simulink model "model"  (R2016a)
(part 3 of 3)

  bus36 : powerlib/Measurements/Load Flow Bus  LConnTagsString=a  Phases=single  Connectors=on one side  ID=bus36  Vbase=220000  Vref=1  Vangle=0  VLF=1  VLFb=1  VLFc=1  angleLF=0  angleLFb=0  angleLFc=0
      settings: AttributesFormatString=|
      | %<ID>
      | %<Vbase>V
      | %<VLF>pu
      | %<angleLF>deg.
      | %<Name>
  bus37 : powerlib/Measurements/Load Flow Bus  LConnTagsString=a  Phases=single  Connectors=on one side  ID=bus37  Vbase=220000  Vref=1  Vangle=0  VLF=1  VLFb=1  VLFc=1  angleLF=0  angleLFb=0  angleLFc=0
      settings: AttributesFormatString=|
      | %<ID>
      | %<Vbase>V
      | %<VLF>pu
      | %<angleLF>deg.
      | %<Name>
  bus38 : powerlib/Measurements/Load Flow Bus  LConnTagsString=a  Phases=single  Connectors=on one side  ID=bus38  Vbase=220000  Vref=1  Vangle=0  VLF=1  VLFb=1  VLFc=1  angleLF=0  angleLFb=0  angleLFc=0
      settings: AttributesFormatString=|
      | %<ID>
      | %<Vbase>V
      | %<VLF>pu
      | %<angleLF>deg.
      | %<Name>
  bus39 : powerlib/Measurements/Load Flow Bus  LConnTagsString=a  Phases=single  Connectors=on one side  ID=bus39  Vbase=220000  Vref=1  Vangle=0  VLF=1  VLFb=1  VLFc=1  angleLF=0  angleLFb=0  angleLFc=0
      settings: AttributesFormatString=|
      | %<ID>
      | %<Vbase>V
      | %<VLF>pu
      | %<angleLF>deg.
      | %<Name>
  bus4 : powerlib/Measurements/Load Flow Bus  LConnTagsString=a  Phases=single  Connectors=on one side  ID=bus4  Vbase=132000  Vref=1  Vangle=0  VLF=1  VLFb=1  VLFc=1  angleLF=0  angleLFb=0  angleLFc=0
      settings: AttributesFormatString=|
      | %<ID>
      | %<Vbase>V
      | %<VLF>pu
      | %<angleLF>deg.
      | %<Name>
  bus40 : powerlib/Measurements/Load Flow Bus  LConnTagsString=a  Phases=single  Connectors=on one side  ID=bus40  Vbase=220000  Vref=1  Vangle=0  VLF=1  VLFb=1  VLFc=1  angleLF=0  angleLFb=0  angleLFc=0
      settings: AttributesFormatString=|
      | %<ID>
      | %<Vbase>V
      | %<VLF>pu
      | %<angleLF>deg.
      | %<Name>
  bus41 : powerlib/Measurements/Load Flow Bus  LConnTagsString=a  Phases=single  Connectors=on one side  ID=bus41  Vbase=220000  Vref=1  Vangle=0  VLF=1  VLFb=1  VLFc=1  angleLF=0  angleLFb=0  angleLFc=0
      settings: AttributesFormatString=|
      | %<ID>
      | %<Vbase>V
      | %<VLF>pu
      | %<angleLF>deg.
      | %<Name>
  bus42 : powerlib/Measurements/Load Flow Bus  LConnTagsString=a  Phases=single  Connectors=on one side  ID=bus42  Vbase=220000  Vref=1  Vangle=0  VLF=1  VLFb=1  VLFc=1  angleLF=0  angleLFb=0  angleLFc=0
      settings: AttributesFormatString=|
      | %<ID>
      | %<Vbase>V
      | %<VLF>pu
      | %<angleLF>deg.
      | %<Name>
  bus43 : powerlib/Measurements/Load Flow Bus  LConnTagsString=a  Phases=single  Connectors=on one side  ID=bus43  Vbase=220000  Vref=1  Vangle=0  VLF=1  VLFb=1  VLFc=1  angleLF=0  angleLFb=0  angleLFc=0
      settings: AttributesFormatString=|
      | %<ID>
      | %<Vbase>V
      | %<VLF>pu
      | %<angleLF>deg.
      | %<Name>
  bus44 : powerlib/Measurements/Load Flow Bus  LConnTagsString=a  Phases=single  Connectors=on one side  ID=bus44  Vbase=220000  Vref=1  Vangle=0  VLF=1  VLFb=1  VLFc=1  angleLF=0  angleLFb=0  angleLFc=0
      settings: AttributesFormatString=|
      | %<ID>
      | %<Vbase>V
      | %<VLF>pu
      | %<angleLF>deg.
      | %<Name>
  bus45 : powerlib/Measurements/Load Flow Bus  LConnTagsString=a  Phases=single  Connectors=on one side  ID=bus45  Vbase=220000  Vref=1  Vangle=0  VLF=1  VLFb=1  VLFc=1  angleLF=0  angleLFb=0  angleLFc=0
      settings: AttributesFormatString=|
      | %<ID>
      | %<Vbase>V
      | %<VLF>pu
      | %<angleLF>deg.
      | %<Name>
  bus46 : powerlib/Measurements/Load Flow Bus  LConnTagsString=a  Phases=single  Connectors=on one side  ID=bus46  Vbase=220000  Vref=1  Vangle=0  VLF=1  VLFb=1  VLFc=1  angleLF=0  angleLFb=0  angleLFc=0
      settings: AttributesFormatString=|
      | %<ID>
      | %<Vbase>V
      | %<VLF>pu
      | %<angleLF>deg.
      | %<Name>
  bus47 : powerlib/Measurements/Load Flow Bus  LConnTagsString=a  Phases=single  Connectors=on one side  ID=bus47  Vbase=220000  Vref=1  Vangle=0  VLF=1  VLFb=1  VLFc=1  angleLF=0  angleLFb=0  angleLFc=0
      settings: AttributesFormatString=|
      | %<ID>
      | %<Vbase>V
      | %<VLF>pu
      | %<angleLF>deg.
      | %<Name>
  bus48 : powerlib/Measurements/Load Flow Bus  LConnTagsString=a  Phases=single  Connectors=on one side  ID=bus48  Vbase=220000  Vref=1  Vangle=0  VLF=1  VLFb=1  VLFc=1  angleLF=0  angleLFb=0  angleLFc=0
      settings: AttributesFormatString=|
      | %<ID>
      | %<Vbase>V
      | %<VLF>pu
      | %<angleLF>deg.
      | %<Name>
  bus49 : powerlib/Measurements/Load Flow Bus  LConnTagsString=a  Phases=single  Connectors=on one side  ID=bus49  Vbase=220000  Vref=1  Vangle=0  VLF=1  VLFb=1  VLFc=1  angleLF=0  angleLFb=0  angleLFc=0
      settings: AttributesFormatString=|
      | %<ID>
      | %<Vbase>V
      | %<VLF>pu
      | %<angleLF>deg.
      | %<Name>
  bus5 : powerlib/Measurements/Load Flow Bus  LConnTagsString=a  Phases=single  Connectors=on one side  ID=bus5  Vbase=132000  Vref=1  Vangle=0  VLF=1  VLFb=1  VLFc=1  angleLF=0  angleLFb=0  angleLFc=0
      settings: AttributesFormatString=|
      | %<ID>
      | %<Vbase>V
      | %<VLF>pu
      | %<angleLF>deg.
      | %<Name>
  bus50 : powerlib/Measurements/Load Flow Bus  LConnTagsString=a  Phases=single  Connectors=on one side  ID=bus50  Vbase=220000  Vref=1  Vangle=0  VLF=1  VLFb=1  VLFc=1  angleLF=0  angleLFb=0  angleLFc=0
      settings: AttributesFormatString=|
      | %<ID>
      | %<Vbase>V
      | %<VLF>pu
      | %<angleLF>deg.
      | %<Name>
  bus51 : powerlib/Measurements/Load Flow Bus  LConnTagsString=a  Phases=single  Connectors=on one side  ID=bus51  Vbase=220000  Vref=1  Vangle=0  VLF=1  VLFb=1  VLFc=1  angleLF=0  angleLFb=0  angleLFc=0
      settings: AttributesFormatString=|
      | %<ID>
      | %<Vbase>V
      | %<VLF>pu
      | %<angleLF>deg.
      | %<Name>
  bus52 : powerlib/Measurements/Load Flow Bus  LConnTagsString=a  Phases=single  Connectors=on one side  ID=bus52  Vbase=220000  Vref=1  Vangle=0  VLF=1  VLFb=1  VLFc=1  angleLF=0  angleLFb=0  angleLFc=0
      settings: AttributesFormatString=|
      | %<ID>
      | %<Vbase>V
      | %<VLF>pu
      | %<angleLF>deg.
      | %<Name>
  bus53 : powerlib/Measurements/Load Flow Bus  LConnTagsString=a  Phases=single  Connectors=on one side  ID=bus53  Vbase=220000  Vref=1  Vangle=0  VLF=1  VLFb=1  VLFc=1  angleLF=0  angleLFb=0  angleLFc=0
      settings: AttributesFormatString=|
      | %<ID>
      | %<Vbase>V
      | %<VLF>pu
      | %<angleLF>deg.
      | %<Name>
  bus54 : powerlib/Measurements/Load Flow Bus  LConnTagsString=a  Phases=single  Connectors=on one side  ID=bus54  Vbase=220000  Vref=1  Vangle=0  VLF=1  VLFb=1  VLFc=1  angleLF=0  angleLFb=0  angleLFc=0
      settings: AttributesFormatString=|
      | %<ID>
      | %<Vbase>V
      | %<VLF>pu
      | %<angleLF>deg.
      | %<Name>
  bus55 : powerlib/Measurements/Load Flow Bus  LConnTagsString=a  Phases=single  Connectors=on one side  ID=bus55  Vbase=220000  Vref=1  Vangle=0  VLF=1  VLFb=1  VLFc=1  angleLF=0  angleLFb=0  angleLFc=0
      settings: AttributesFormatString=|
      | %<ID>
      | %<Vbase>V
      | %<VLF>pu
      | %<angleLF>deg.
      | %<Name>
  bus56 : powerlib/Measurements/Load Flow Bus  LConnTagsString=a  Phases=single  Connectors=on one side  ID=bus56  Vbase=220000  Vref=1  Vangle=0  VLF=1  VLFb=1  VLFc=1  angleLF=0  angleLFb=0  angleLFc=0
      settings: AttributesFormatString=|
      | %<ID>
      | %<Vbase>V
      | %<VLF>pu
      | %<angleLF>deg.
      | %<Name>
  bus57 : powerlib/Measurements/Load Flow Bus  LConnTagsString=a  Phases=single  Connectors=on one side  ID=bus57  Vbase=220000  Vref=1  Vangle=0  VLF=1  VLFb=1  VLFc=1  angleLF=0  angleLFb=0  angleLFc=0
      settings: AttributesFormatString=|
      | %<ID>
      | %<Vbase>V
      | %<VLF>pu
      | %<angleLF>deg.
      | %<Name>
  bus58 : powerlib/Measurements/Load Flow Bus  LConnTagsString=a  Phases=single  Connectors=on one side  ID=bus58  Vbase=220000  Vref=1  Vangle=0  VLF=1  VLFb=1  VLFc=1  angleLF=0  angleLFb=0  angleLFc=0
      settings: AttributesFormatString=|
      | %<ID>
      | %<Vbase>V
      | %<VLF>pu
      | %<angleLF>deg.
      | %<Name>
  bus59 : powerlib/Measurements/Load Flow Bus  LConnTagsString=a  Phases=single  Connectors=on one side  ID=bus59  Vbase=220000  Vref=1  Vangle=0  VLF=1  VLFb=1  VLFc=1  angleLF=0  angleLFb=0  angleLFc=0
      settings: AttributesFormatString=|
      | %<ID>
      | %<Vbase>V
      | %<VLF>pu
      | %<angleLF>deg.
      | %<Name>
  bus6 : powerlib/Measurements/Load Flow Bus  LConnTagsString=a  Phases=single  Connectors=on one side  ID=bus6  Vbase=132000  Vref=1  Vangle=0  VLF=1  VLFb=1  VLFc=1  angleLF=0  angleLFb=0  angleLFc=0
      settings: AttributesFormatString=|
      | %<ID>
      | %<Vbase>V
      | %<VLF>pu
      | %<angleLF>deg.
      | %<Name>
  bus60 : powerlib/Measurements/Load Flow Bus  LConnTagsString=a  Phases=single  Connectors=on one side  ID=bus60  Vbase=220000  Vref=1  Vangle=0  VLF=1  VLFb=1  VLFc=1  angleLF=0  angleLFb=0  angleLFc=0
      settings: AttributesFormatString=|
      | %<ID>
      | %<Vbase>V
      | %<VLF>pu
      | %<angleLF>deg.
      | %<Name>
  bus61 : powerlib/Measurements/Load Flow Bus  LConnTagsString=a  Phases=single  Connectors=on one side  ID=bus61  Vbase=220000  Vref=1  Vangle=0  VLF=1  VLFb=1  VLFc=1  angleLF=0  angleLFb=0  angleLFc=0
      settings: AttributesFormatString=|
      | %<ID>
      | %<Vbase>V
      | %<VLF>pu
      | %<angleLF>deg.
      | %<Name>
  bus62 : powerlib/Measurements/Load Flow Bus  LConnTagsString=a  Phases=single  Connectors=on one side  ID=bus62  Vbase=220000  Vref=1  Vangle=0  VLF=1  VLFb=1  VLFc=1  angleLF=0  angleLFb=0  angleLFc=0
      settings: AttributesFormatString=|
      | %<ID>
      | %<Vbase>V
      | %<VLF>pu
      | %<angleLF>deg.
      | %<Name>
  bus63 : powerlib/Measurements/Load Flow Bus  LConnTagsString=a  Phases=single  Connectors=on one side  ID=bus63  Vbase=220000  Vref=1  Vangle=0  VLF=1  VLFb=1  VLFc=1  angleLF=0  angleLFb=0  angleLFc=0
      settings: AttributesFormatString=|
      | %<ID>
      | %<Vbase>V
      | %<VLF>pu
      | %<angleLF>deg.
      | %<Name>
  bus64 : powerlib/Measurements/Load Flow Bus  LConnTagsString=a  Phases=single  Connectors=on one side  ID=bus64  Vbase=220000  Vref=1  Vangle=0  VLF=1  VLFb=1  VLFc=1  angleLF=0  angleLFb=0  angleLFc=0
      settings: AttributesFormatString=|
      | %<ID>
      | %<Vbase>V
      | %<VLF>pu
      | %<angleLF>deg.
      | %<Name>
  bus65 : powerlib/Measurements/Load Flow Bus  LConnTagsString=a  Phases=single  Connectors=on one side  ID=bus65  Vbase=220000  Vref=1  Vangle=0  VLF=1  VLFb=1  VLFc=1  angleLF=0  angleLFb=0  angleLFc=0
      settings: AttributesFormatString=|
      | %<ID>
      | %<Vbase>V
      | %<VLF>pu
      | %<angleLF>deg.
      | %<Name>
  bus66 : powerlib/Measurements/Load Flow Bus  LConnTagsString=a  Phases=single  Connectors=on one side  ID=bus66  Vbase=220000  Vref=1  Vangle=0  VLF=1  VLFb=1  VLFc=1  angleLF=0  angleLFb=0  angleLFc=0
      settings: AttributesFormatString=|
      | %<ID>
      | %<Vbase>V
      | %<VLF>pu
      | %<angleLF>deg.
      | %<Name>
  bus67 : powerlib/Measurements/Load Flow Bus  LConnTagsString=a  Phases=single  Connectors=on one side  ID=bus67  Vbase=220000  Vref=1  Vangle=0  VLF=1  VLFb=1  VLFc=1  angleLF=0  angleLFb=0  angleLFc=0
      settings: AttributesFormatString=|
      | %<ID>
      | %<Vbase>V
      | %<VLF>pu
      | %<angleLF>deg.
      | %<Name>
  bus68 : powerlib/Measurements/Load Flow Bus  LConnTagsString=a  Phases=single  Connectors=on one side  ID=bus68  Vbase=220000  Vref=1  Vangle=0  VLF=1  VLFb=1  VLFc=1  angleLF=0  angleLFb=0  angleLFc=0
      settings: AttributesFormatString=|
      | %<ID>
      | %<Vbase>V
      | %<VLF>pu
      | %<angleLF>deg.
      | %<Name>
  bus69 : powerlib/Measurements/Load Flow Bus  LConnTagsString=a  Phases=single  Connectors=on one side  ID=bus69  Vbase=220000  Vref=1  Vangle=0  VLF=1  VLFb=1  VLFc=1  angleLF=0  angleLFb=0  angleLFc=0
      settings: AttributesFormatString=|
      | %<ID>
      | %<Vbase>V
      | %<VLF>pu
      | %<angleLF>deg.
      | %<Name>
  bus7 : powerlib/Measurements/Load Flow Bus  LConnTagsString=a  Phases=single  Connectors=on one side  ID=bus7  Vbase=132000  Vref=1  Vangle=0  VLF=1  VLFb=1  VLFc=1  angleLF=0  angleLFb=0  angleLFc=0
      settings: AttributesFormatString=|
      | %<ID>
      | %<Vbase>V
      | %<VLF>pu
      | %<angleLF>deg.
      | %<Name>
  bus70 : powerlib/Measurements/Load Flow Bus  LConnTagsString=a  Phases=single  Connectors=on one side  ID=bus70  Vbase=220000  Vref=1  Vangle=0  VLF=1  VLFb=1  VLFc=1  angleLF=0  angleLFb=0  angleLFc=0
      settings: AttributesFormatString=|
      | %<ID>
      | %<Vbase>V
      | %<VLF>pu
      | %<angleLF>deg.
      | %<Name>
  bus71 : powerlib/Measurements/Load Flow Bus  LConnTagsString=a  Phases=single  Connectors=on one side  ID=bus71  Vbase=220000  Vref=1  Vangle=0  VLF=1  VLFb=1  VLFc=1  angleLF=0  angleLFb=0  angleLFc=0
      settings: AttributesFormatString=|
      | %<ID>
      | %<Vbase>V
      | %<VLF>pu
      | %<angleLF>deg.
      | %<Name>
  bus72 : powerlib/Measurements/Load Flow Bus  LConnTagsString=a  Phases=single  Connectors=on one side  ID=bus72  Vbase=220000  Vref=1  Vangle=0  VLF=1  VLFb=1  VLFc=1  angleLF=0  angleLFb=0  angleLFc=0
      settings: AttributesFormatString=|
      | %<ID>
      | %<Vbase>V
      | %<VLF>pu
      | %<angleLF>deg.
      | %<Name>
  bus73 : powerlib/Measurements/Load Flow Bus  LConnTagsString=a  Phases=single  Connectors=on one side  ID=bus73  Vbase=220000  Vref=1  Vangle=0  VLF=1  VLFb=1  VLFc=1  angleLF=0  angleLFb=0  angleLFc=0
      settings: AttributesFormatString=|
      | %<ID>
      | %<Vbase>V
      | %<VLF>pu
      | %<angleLF>deg.
      | %<Name>
  bus74 : powerlib/Measurements/Load Flow Bus  LConnTagsString=a  Phases=single  Connectors=on one side  ID=bus74  Vbase=220000  Vref=1  Vangle=0  VLF=1  VLFb=1  VLFc=1  angleLF=0  angleLFb=0  angleLFc=0
      settings: AttributesFormatString=|
      | %<ID>
      | %<Vbase>V
      | %<VLF>pu
      | %<angleLF>deg.
      | %<Name>
  bus75 : powerlib/Measurements/Load Flow Bus  LConnTagsString=a  Phases=single  Connectors=on one side  ID=bus75  Vbase=220000  Vref=1  Vangle=0  VLF=1  VLFb=1  VLFc=1  angleLF=0  angleLFb=0  angleLFc=0
      settings: AttributesFormatString=|
      | %<ID>
      | %<Vbase>V
      | %<VLF>pu
      | %<angleLF>deg.
      | %<Name>
  bus76 : powerlib/Measurements/Load Flow Bus  LConnTagsString=a  Phases=single  Connectors=on one side  ID=bus76  Vbase=220000  Vref=1  Vangle=0  VLF=1  VLFb=1  VLFc=1  angleLF=0  angleLFb=0  angleLFc=0
      settings: AttributesFormatString=|
      | %<ID>
      | %<Vbase>V
      | %<VLF>pu
      | %<angleLF>deg.
      | %<Name>
  bus77 : powerlib/Measurements/Load Flow Bus  LConnTagsString=a  Phases=single  Connectors=on one side  ID=bus77  Vbase=220000  Vref=1  Vangle=0  VLF=1  VLFb=1  VLFc=1  angleLF=0  angleLFb=0  angleLFc=0
      settings: AttributesFormatString=|
      | %<ID>
      | %<Vbase>V
      | %<VLF>pu
      | %<angleLF>deg.
      | %<Name>
  bus78 : powerlib/Measurements/Load Flow Bus  LConnTagsString=a  Phases=single  Connectors=on one side  ID=bus78  Vbase=220000  Vref=1  Vangle=0  VLF=1  VLFb=1  VLFc=1  angleLF=0  angleLFb=0  angleLFc=0
      settings: AttributesFormatString=|
      | %<ID>
      | %<Vbase>V
      | %<VLF>pu
      | %<angleLF>deg.
      | %<Name>
  bus79 : powerlib/Measurements/Load Flow Bus  LConnTagsString=a  Phases=single  Connectors=on one side  ID=bus79  Vbase=220000  Vref=1  Vangle=0  VLF=1  VLFb=1  VLFc=1  angleLF=0  angleLFb=0  angleLFc=0
      settings: AttributesFormatString=|
      | %<ID>
      | %<Vbase>V
      | %<VLF>pu
      | %<angleLF>deg.
      | %<Name>
  bus8 : powerlib/Measurements/Load Flow Bus  LConnTagsString=a  Phases=single  Connectors=on one side  ID=bus8  Vbase=132000  Vref=1  Vangle=0  VLF=1  VLFb=1  VLFc=1  angleLF=0  angleLFb=0  angleLFc=0
      settings: AttributesFormatString=|
      | %<ID>
      | %<Vbase>V
      | %<VLF>pu
      | %<angleLF>deg.
      | %<Name>
  bus80 : powerlib/Measurements/Load Flow Bus  LConnTagsString=a  Phases=single  Connectors=on one side  ID=bus80  Vbase=220000  Vref=1  Vangle=0  VLF=1  VLFb=1  VLFc=1  angleLF=0  angleLFb=0  angleLFc=0
      settings: AttributesFormatString=|
      | %<ID>
      | %<Vbase>V
      | %<VLF>pu
      | %<angleLF>deg.
      | %<Name>
  bus81 : powerlib/Measurements/Load Flow Bus  LConnTagsString=a  Phases=single  Connectors=on one side  ID=bus81  Vbase=220000  Vref=1  Vangle=0  VLF=1  VLFb=1  VLFc=1  angleLF=0  angleLFb=0  angleLFc=0
      settings: AttributesFormatString=|
      | %<ID>
      | %<Vbase>V
      | %<VLF>pu
      | %<angleLF>deg.
      | %<Name>
  bus82 : powerlib/Measurements/Load Flow Bus  LConnTagsString=a  Phases=single  Connectors=on one side  ID=bus82  Vbase=220000  Vref=1  Vangle=0  VLF=1  VLFb=1  VLFc=1  angleLF=0  angleLFb=0  angleLFc=0
      settings: AttributesFormatString=|
      | %<ID>
      | %<Vbase>V
      | %<VLF>pu
      | %<angleLF>deg.
      | %<Name>
  bus83 : powerlib/Measurements/Load Flow Bus  LConnTagsString=a  Phases=single  Connectors=on one side  ID=bus83  Vbase=220000  Vref=1  Vangle=0  VLF=1  VLFb=1  VLFc=1  angleLF=0  angleLFb=0  angleLFc=0
      settings: AttributesFormatString=|
      | %<ID>
      | %<Vbase>V
      | %<VLF>pu
      | %<angleLF>deg.
      | %<Name>
  bus84 : powerlib/Measurements/Load Flow Bus  LConnTagsString=a  Phases=single  Connectors=on one side  ID=bus84  Vbase=220000  Vref=1  Vangle=0  VLF=1  VLFb=1  VLFc=1  angleLF=0  angleLFb=0  angleLFc=0
      settings: AttributesFormatString=|
      | %<ID>
      | %<Vbase>V
      | %<VLF>pu
      | %<angleLF>deg.
      | %<Name>
  bus85 : powerlib/Measurements/Load Flow Bus  LConnTagsString=a  Phases=single  Connectors=on one side  ID=bus85  Vbase=220000  Vref=1  Vangle=0  VLF=1  VLFb=1  VLFc=1  angleLF=0  angleLFb=0  angleLFc=0
      settings: AttributesFormatString=|
      | %<ID>
      | %<Vbase>V
      | %<VLF>pu
      | %<angleLF>deg.
      | %<Name>
  bus86 : powerlib/Measurements/Load Flow Bus  LConnTagsString=a  Phases=single  Connectors=on one side  ID=bus86  Vbase=220000  Vref=1  Vangle=0  VLF=1  VLFb=1  VLFc=1  angleLF=0  angleLFb=0  angleLFc=0
      settings: AttributesFormatString=|
      | %<ID>
      | %<Vbase>V
      | %<VLF>pu
      | %<angleLF>deg.
      | %<Name>
  bus87 : powerlib/Measurements/Load Flow Bus  LConnTagsString=a  Phases=single  Connectors=on one side  ID=bus87  Vbase=220000  Vref=1  Vangle=0  VLF=1  VLFb=1  VLFc=1  angleLF=0  angleLFb=0  angleLFc=0
      settings: AttributesFormatString=|
      | %<ID>
      | %<Vbase>V
      | %<VLF>pu
      | %<angleLF>deg.
      | %<Name>
  bus88 : powerlib/Measurements/Load Flow Bus  LConnTagsString=a  Phases=single  Connectors=on one side  ID=bus88  Vbase=220000  Vref=1  Vangle=0  VLF=1  VLFb=1  VLFc=1  angleLF=0  angleLFb=0  angleLFc=0
      settings: AttributesFormatString=|
      | %<ID>
      | %<Vbase>V
      | %<VLF>pu
      | %<angleLF>deg.
      | %<Name>
  bus89 : powerlib/Measurements/Load Flow Bus  LConnTagsString=a  Phases=single  Connectors=on one side  ID=bus89  Vbase=220000  Vref=1  Vangle=0  VLF=1  VLFb=1  VLFc=1  angleLF=0  angleLFb=0  angleLFc=0
      settings: AttributesFormatString=|
      | %<ID>
      | %<Vbase>V
      | %<VLF>pu
      | %<angleLF>deg.
      | %<Name>
  bus9 : powerlib/Measurements/Load Flow Bus  LConnTagsString=a  Phases=single  Connectors=on one side  ID=bus9  Vbase=132000  Vref=1  Vangle=0  VLF=1  VLFb=1  VLFc=1  angleLF=0  angleLFb=0  angleLFc=0
      settings: AttributesFormatString=|
      | %<ID>
      | %<Vbase>V
      | %<VLF>pu
      | %<angleLF>deg.
      | %<Name>
  bus90 : powerlib/Measurements/Load Flow Bus  LConnTagsString=a  Phases=single  Connectors=on one side  ID=bus90  Vbase=220000  Vref=1  Vangle=0  VLF=1  VLFb=1  VLFc=1  angleLF=0  angleLFb=0  angleLFc=0
      settings: AttributesFormatString=|
      | %<ID>
      | %<Vbase>V
      | %<VLF>pu
      | %<angleLF>deg.
      | %<Name>
  bus91 : powerlib/Measurements/Load Flow Bus  LConnTagsString=a  Phases=single  Connectors=on one side  ID=bus91  Vbase=220000  Vref=1  Vangle=0  VLF=1  VLFb=1  VLFc=1  angleLF=0  angleLFb=0  angleLFc=0
      settings: AttributesFormatString=|
      | %<ID>
      | %<Vbase>V
      | %<VLF>pu
      | %<angleLF>deg.
      | %<Name>
  bus92 : powerlib/Measurements/Load Flow Bus  LConnTagsString=a  Phases=single  Connectors=on one side  ID=bus92  Vbase=220000  Vref=1  Vangle=0  VLF=1  VLFb=1  VLFc=1  angleLF=0  angleLFb=0  angleLFc=0
      settings: AttributesFormatString=|
      | %<ID>
      | %<Vbase>V
      | %<VLF>pu
      | %<angleLF>deg.
      | %<Name>
  bus93 : powerlib/Measurements/Load Flow Bus  LConnTagsString=a  Phases=single  Connectors=on one side  ID=bus93  Vbase=220000  Vref=1  Vangle=0  VLF=1  VLFb=1  VLFc=1  angleLF=0  angleLFb=0  angleLFc=0
      settings: AttributesFormatString=|
      | %<ID>
      | %<Vbase>V
      | %<VLF>pu
      | %<angleLF>deg.
      | %<Name>
  bus94 : powerlib/Measurements/Load Flow Bus  LConnTagsString=a  Phases=single  Connectors=on one side  ID=bus94  Vbase=220000  Vref=1  Vangle=0  VLF=1  VLFb=1  VLFc=1  angleLF=0  angleLFb=0  angleLFc=0
      settings: AttributesFormatString=|
      | %<ID>
      | %<Vbase>V
      | %<VLF>pu
      | %<angleLF>deg.
      | %<Name>
  bus95 : powerlib/Measurements/Load Flow Bus  LConnTagsString=a  Phases=single  Connectors=on one side  ID=bus95  Vbase=220000  Vref=1  Vangle=0  VLF=1  VLFb=1  VLFc=1  angleLF=0  angleLFb=0  angleLFc=0
      settings: AttributesFormatString=|
      | %<ID>
      | %<Vbase>V
      | %<VLF>pu
      | %<angleLF>deg.
      | %<Name>
  bus96 : powerlib/Measurements/Load Flow Bus  LConnTagsString=a  Phases=single  Connectors=on one side  ID=bus96  Vbase=220000  Vref=1  Vangle=0  VLF=1  VLFb=1  VLFc=1  angleLF=0  angleLFb=0  angleLFc=0
      settings: AttributesFormatString=|
      | %<ID>
      | %<Vbase>V
      | %<VLF>pu
      | %<angleLF>deg.
      | %<Name>
  bus97 : powerlib/Measurements/Load Flow Bus  LConnTagsString=a  Phases=single  Connectors=on one side  ID=bus97  Vbase=220000  Vref=1  Vangle=0  VLF=1  VLFb=1  VLFc=1  angleLF=0  angleLFb=0  angleLFc=0
      settings: AttributesFormatString=|
      | %<ID>
      | %<Vbase>V
      | %<VLF>pu
      | %<angleLF>deg.
      | %<Name>
  bus98 : powerlib/Measurements/Load Flow Bus  LConnTagsString=a  Phases=single  Connectors=on one side  ID=bus98  Vbase=220000  Vref=1  Vangle=0  VLF=1  VLFb=1  VLFc=1  angleLF=0  angleLFb=0  angleLFc=0
      settings: AttributesFormatString=|
      | %<ID>
      | %<Vbase>V
      | %<VLF>pu
      | %<angleLF>deg.
      | %<Name>
  bus99 : powerlib/Measurements/Load Flow Bus  LConnTagsString=a  Phases=single  Connectors=on one side  ID=bus99  Vbase=220000  Vref=1  Vangle=0  VLF=1  VLFb=1  VLFc=1  angleLF=0  angleLFb=0  angleLFc=0
      settings: AttributesFormatString=|
      | %<ID>
      | %<Vbase>V
      | %<VLF>pu
      | %<angleLF>deg.
      | %<Name>
  powergui : powerlib/powergui  Priority=1  SimulationMode=Phasor  SolverType=Tustin/Backward Euler (TBE)  SampleTime=50e-6  frequency=50  SPID=off  DisableSnubberDevices=off  DisableRonSwitches=off  DisableVfSwitches=off  SwTol=0  DisplayEquations=off  Interpol=off  ExternalGateDelay=off  methode=off  Ts=10  FunctionMessages=off  echomessages=off  HookPort=off  EnableUseOfTLC=off  x0status=blocks  frequencyindice=50  Pbase=3000e6  ErrMax=0.0001  Iterations=50  UnitsV=V  UnitsW=W  buscounter=0  RestoreLinks=warning  ResistiveCurrentMeasurement=off  Frange=[0:2:500]  Ylog=off  Xlog=on  ShowGrid=off  save=off  variable=ZData  structure=0  ZoomFFT=off  StartTime=0.0  cycles=1  DisplayStyle=1  fundamental=60  FreqAxis=off  MaxFrequency=1000  frequencyindicesteady=1  RmsSteady=1  display=off
  connections:
  _CN_426998273_132000_CN_426825819_132000/LConn1 -- T_426998273__/RConn1 -- _CN_426998273_132000_CN_102788377_132000/LConn1 -- _CN_426998273_132000_CN_112984533_132000/LConn1 -- _CN_426998273_132000_CN_113004375_132000/LConn1 -- _CN_426998273_132000_CN_219583075_132000/LConn1 -- L_426998273/LConn1
  _CN_426998273_132000_CN_426825819_132000/LConn2 -- T_426998273__/RConn2 -- _CN_426998273_132000_CN_102788377_132000/LConn2 -- _CN_426998273_132000_CN_112984533_132000/LConn2 -- _CN_426998273_132000_CN_113004375_132000/LConn2 -- _CN_426998273_132000_CN_219583075_132000/LConn2 -- L_426998273/LConn2
  _CN_426998273_132000_CN_426825819_132000/LConn3 -- T_426998273__/RConn3 -- _CN_426998273_132000_CN_102788377_132000/LConn3 -- _CN_426998273_132000_CN_112984533_132000/LConn3 -- _CN_426998273_132000_CN_113004375_132000/LConn3 -- _CN_426998273_132000_CN_219583075_132000/LConn3 -- L_426998273/LConn3 -- bus1/LConn1
  _CN_426998273_132000_CN_426825819_132000/RConn1 -- T_426825819__/LConn1 -- _CN_426825819_132000_CN_219583075_132000/LConn1
  _CN_426998273_132000_CN_426825819_132000/RConn2 -- T_426825819__/LConn2 -- _CN_426825819_132000_CN_219583075_132000/LConn2
  _CN_426998273_132000_CN_426825819_132000/RConn3 -- T_426825819__/LConn3 -- _CN_426825819_132000_CN_219583075_132000/LConn3 -- bus2/LConn1
  T_102788377_132000;66000_/LConn1 -- _CN_426998273_132000_CN_102788377_132000/RConn1
  T_102788377_132000;66000_/LConn2 -- _CN_426998273_132000_CN_102788377_132000/RConn2
  _CN_426998273_132000_CN_102788377_132000/RConn3 -- T_102788377_132000;66000_/LConn3 -- bus3/LConn1
  _CN_426998273_132000_CN_112984533_132000/RConn1 -- T_112984533_132000_/LConn1 -- _CN_230637780_132000_CN_112984533_132000/LConn1
  _CN_426998273_132000_CN_112984533_132000/RConn2 -- T_112984533_132000_/LConn2 -- _CN_230637780_132000_CN_112984533_132000/LConn2
  _CN_426998273_132000_CN_112984533_132000/RConn3 -- T_112984533_132000_/LConn3 -- _CN_230637780_132000_CN_112984533_132000/LConn3 -- bus4/LConn1
  T_113004375_132000_/LConn1 -- _CN_426998273_132000_CN_113004375_132000/RConn1
  T_113004375_132000_/LConn2 -- _CN_426998273_132000_CN_113004375_132000/RConn2
  _CN_426998273_132000_CN_113004375_132000/RConn3 -- T_113004375_132000_/LConn3 -- bus5/LConn1
  _CN_426998273_132000_CN_219583075_132000/RConn1 -- T_219583075_132000_/LConn1 -- _CN_219583075_132000_CN_130440404_132000/LConn1 -- _CN_426825819_132000_CN_219583075_132000/RConn1
  _CN_426998273_132000_CN_219583075_132000/RConn2 -- T_219583075_132000_/LConn2 -- _CN_219583075_132000_CN_130440404_132000/LConn2 -- _CN_426825819_132000_CN_219583075_132000/RConn2
  _CN_426998273_132000_CN_219583075_132000/RConn3 -- T_219583075_132000_/LConn3 -- _CN_219583075_132000_CN_130440404_132000/LConn3 -- bus6/LConn1 -- _CN_426825819_132000_CN_219583075_132000/RConn3
  T_263541774__/LConn1 -- _CN_263541774_132000_CN_117393191_132000/LConn1
  T_263541774__/LConn2 -- _CN_263541774_132000_CN_117393191_132000/LConn2
  _CN_263541774_132000_CN_117393191_132000/LConn3 -- T_263541774__/LConn3 -- bus7/LConn1
  _CN_263541774_132000_CN_117393191_132000/RConn1 -- T_117393191_500000;220000;132000_/RConn4 -- _CN_263541777_132000_CN_117393191_132000/LConn1 -- L_117393191/LConn1
  _CN_263541774_132000_CN_117393191_132000/RConn2 -- T_117393191_500000;220000;132000_/RConn5 -- _CN_263541777_132000_CN_117393191_132000/LConn2 -- L_117393191/LConn2
  _CN_263541774_132000_CN_117393191_132000/RConn3 -- T_117393191_500000;220000;132000_/RConn6 -- _CN_263541777_132000_CN_117393191_132000/LConn3 -- L_117393191/LConn3 -- bus8/LConn1
  T_263541777__/LConn1 -- _CN_263541777_132000_CN_117393191_132000/RConn1
  T_263541777__/LConn2 -- _CN_263541777_132000_CN_117393191_132000/RConn2
  _CN_263541777_132000_CN_117393191_132000/RConn3 -- T_263541777__/LConn3 -- bus9/LConn1
  _CN_115491527_132000_CN_117328910_132000/LConn1 -- T_115491527_500000;220000;132000_/RConn4 -- _CN_115491527_132000_CN_115498840_132000/LConn1 -- _CN_115491527_132000_CN_213203947_132000/LConn1 -- L_115491527/LConn1
  _CN_115491527_132000_CN_117328910_132000/LConn2 -- T_115491527_500000;220000;132000_/RConn5 -- _CN_115491527_132000_CN_115498840_132000/LConn2 -- _CN_115491527_132000_CN_213203947_132000/LConn2 -- L_115491527/LConn2
  _CN_115491527_132000_CN_117328910_132000/LConn3 -- T_115491527_500000;220000;132000_/RConn6 -- _CN_115491527_132000_CN_115498840_132000/LConn3 -- _CN_115491527_132000_CN_213203947_132000/LConn3 -- L_115491527/LConn3 -- bus10/LConn1
  T_117328910__/LConn1 -- _CN_115491527_132000_CN_117328910_132000/RConn1
  T_117328910__/LConn2 -- _CN_115491527_132000_CN_117328910_132000/RConn2
  _CN_115491527_132000_CN_117328910_132000/RConn3 -- T_117328910__/LConn3 -- bus11/LConn1
  _CN_115491527_132000_CN_115498840_132000/RConn1 -- T_115498840__/RConn1 -- L_115498840/LConn1
  _CN_115491527_132000_CN_115498840_132000/RConn2 -- T_115498840__/RConn2 -- L_115498840/LConn2
  _CN_115491527_132000_CN_115498840_132000/RConn3 -- T_115498840__/RConn3 -- L_115498840/LConn3 -- bus12/LConn1
  _CN_115491527_132000_CN_213203947_132000/RConn1 -- T_213203947_132000;66000_/LConn1 -- _CN_116612828_132000_CN_213203947_132000/LConn1 -- _CN_213203947_132000_CN_213203948_132000/LConn1
  _CN_115491527_132000_CN_213203947_132000/RConn2 -- T_213203947_132000;66000_/LConn2 -- _CN_116612828_132000_CN_213203947_132000/LConn2 -- _CN_213203947_132000_CN_213203948_132000/LConn2
  _CN_115491527_132000_CN_213203947_132000/RConn3 -- T_213203947_132000;66000_/LConn3 -- _CN_116612828_132000_CN_213203947_132000/LConn3 -- _CN_213203947_132000_CN_213203948_132000/LConn3 -- bus13/LConn1
  T_130440397_132000_/LConn1 -- _CN_130440397_132000_CN_130440404_132000/LConn1
  T_130440397_132000_/LConn2 -- _CN_130440397_132000_CN_130440404_132000/LConn2
  _CN_130440397_132000_CN_130440404_132000/LConn3 -- T_130440397_132000_/LConn3 -- bus14/LConn1
  _CN_130440397_132000_CN_130440404_132000/RConn1 -- T_130440404_132000_/LConn1 -- _CN_116612828_132000_CN_130440404_132000/LConn1 -- _CN_219583075_132000_CN_130440404_132000/RConn1
  _CN_130440397_132000_CN_130440404_132000/RConn2 -- T_130440404_132000_/LConn2 -- _CN_116612828_132000_CN_130440404_132000/LConn2 -- _CN_219583075_132000_CN_130440404_132000/RConn2
  _CN_130440397_132000_CN_130440404_132000/RConn3 -- T_130440404_132000_/LConn3 -- _CN_116612828_132000_CN_130440404_132000/LConn3 -- _CN_219583075_132000_CN_130440404_132000/RConn3 -- bus15/LConn1
  T_230637780_132000_/LConn1 -- _CN_230637780_132000_CN_112984533_132000/RConn1
  T_230637780_132000_/LConn2 -- _CN_230637780_132000_CN_112984533_132000/RConn2
  _CN_230637780_132000_CN_112984533_132000/RConn3 -- T_230637780_132000_/LConn3 -- bus16/LConn1
  _CN_116612828_132000_CN_213203947_132000/RConn1 -- T_116612828_220000_/LConn1 -- _CN_116612828_132000_CN_130440404_132000/RConn1
  _CN_116612828_132000_CN_213203947_132000/RConn2 -- T_116612828_220000_/LConn2 -- _CN_116612828_132000_CN_130440404_132000/RConn2
  _CN_116612828_132000_CN_213203947_132000/RConn3 -- T_116612828_220000_/LConn3 -- _CN_116612828_132000_CN_130440404_132000/RConn3 -- bus17/LConn1
  _CN_213203947_132000_CN_213203948_132000/RConn1 -- T_213203948_220000;132000;66000_/RConn1 -- L_213203948/LConn1
  _CN_213203947_132000_CN_213203948_132000/RConn2 -- T_213203948_220000;132000;66000_/RConn2 -- L_213203948/LConn2
  _CN_213203947_132000_CN_213203948_132000/RConn3 -- T_213203948_220000;132000;66000_/RConn3 -- L_213203948/LConn3 -- bus18/LConn1
  _CN_426998273_220000_CN_130435119_220000/LConn1 -- T_426998273__/LConn1 -- _CN_426998273_220000_CN_112984529_220000/LConn1 -- _CN_426998273_220000_CN_263290997_220000/LConn1
  _CN_426998273_220000_CN_130435119_220000/LConn2 -- T_426998273__/LConn2 -- _CN_426998273_220000_CN_112984529_220000/LConn2 -- _CN_426998273_220000_CN_263290997_220000/LConn2
  _CN_426998273_220000_CN_130435119_220000/LConn3 -- T_426998273__/LConn3 -- _CN_426998273_220000_CN_112984529_220000/LConn3 -- _CN_426998273_220000_CN_263290997_220000/LConn3 -- bus19/LConn1
  _CN_426998273_220000_CN_130435119_220000/RConn1 -- T_130435119_220000;66000_/LConn1 -- _CN_130435119_220000_CN_219295621_220000/LConn1 -- _CN_130435119_220000_CN_219583071_220000/LConn1
  _CN_426998273_220000_CN_130435119_220000/RConn2 -- T_130435119_220000;66000_/LConn2 -- _CN_130435119_220000_CN_219295621_220000/LConn2 -- _CN_130435119_220000_CN_219583071_220000/LConn2
  _CN_426998273_220000_CN_130435119_220000/RConn3 -- T_130435119_220000;66000_/LConn3 -- _CN_130435119_220000_CN_219295621_220000/LConn3 -- bus20/LConn1 -- _CN_130435119_220000_CN_219583071_220000/LConn3
  G_112984529_/RConn1 -- _CN_426998273_220000_CN_112984529_220000/RConn1
  G_112984529_/RConn2 -- _CN_426998273_220000_CN_112984529_220000/RConn2
  _CN_426998273_220000_CN_112984529_220000/RConn3 -- G_112984529_/RConn3 -- bus21/LConn1
  _CN_426998273_220000_CN_263290997_220000/RConn1 -- T_263290997_220000;66000_/LConn1 -- _CN_263290997_220000_CN_263365083_220000/LConn1 -- _CN_213211662_220000_CN_263290997_220000/LConn1
  _CN_426998273_220000_CN_263290997_220000/RConn2 -- T_263290997_220000;66000_/LConn2 -- _CN_263290997_220000_CN_263365083_220000/LConn2 -- _CN_213211662_220000_CN_263290997_220000/LConn2
  _CN_426998273_220000_CN_263290997_220000/RConn3 -- T_263290997_220000;66000_/LConn3 -- _CN_263290997_220000_CN_263365083_220000/LConn3 -- bus22/LConn1 -- _CN_213211662_220000_CN_263290997_220000/LConn3
  _CN_218972674_220000_CN_128182735_220000/LConn1 -- T_218972674__/RConn1 -- L_218972674/LConn1
  _CN_218972674_220000_CN_128182735_220000/LConn2 -- T_218972674__/RConn2 -- L_218972674/LConn2
  _CN_218972674_220000_CN_128182735_220000/LConn3 -- T_218972674__/RConn3 -- L_218972674/LConn3 -- bus23/LConn1
  _CN_218972674_220000_CN_128182735_220000/RConn1 -- T_128182735_220000_/LConn1 -- _CN_128123911_220000_CN_128182735_220000/LConn1 -- _CN_128129616_220000_CN_128182735_220000/LConn1
  _CN_218972674_220000_CN_128182735_220000/RConn2 -- T_128182735_220000_/LConn2 -- _CN_128123911_220000_CN_128182735_220000/LConn2 -- _CN_128129616_220000_CN_128182735_220000/LConn2
  _CN_218972674_220000_CN_128182735_220000/RConn3 -- T_128182735_220000_/LConn3 -- _CN_128123911_220000_CN_128182735_220000/LConn3 -- _CN_128129616_220000_CN_128182735_220000/LConn3 -- bus24/LConn1
  T_98390022_220000;66000_/LConn1 -- _CN_98390022_220000_CN_93650324_220000/LConn1
  T_98390022_220000;66000_/LConn2 -- _CN_98390022_220000_CN_93650324_220000/LConn2
  _CN_98390022_220000_CN_93650324_220000/LConn3 -- T_98390022_220000;66000_/LConn3 -- bus25/LConn1
  _CN_98390022_220000_CN_93650324_220000/RConn1 -- T_93650324_220000_/LConn1 -- _CN_93699965_220000_CN_93650324_220000/LConn1 -- _CN_93650324_220000_CN_214806696_220000/LConn1 -- _CN_218898508_220000_CN_93650324_220000/LConn1
  _CN_98390022_220000_CN_93650324_220000/RConn2 -- T_93650324_220000_/LConn2 -- _CN_93699965_220000_CN_93650324_220000/LConn2 -- _CN_93650324_220000_CN_214806696_220000/LConn2 -- _CN_218898508_220000_CN_93650324_220000/LConn2
  _CN_98390022_220000_CN_93650324_220000/RConn3 -- T_93650324_220000_/LConn3 -- _CN_93699965_220000_CN_93650324_220000/LConn3 -- _CN_93650324_220000_CN_214806696_220000/LConn3 -- bus26/LConn1 -- _CN_218898508_220000_CN_93650324_220000/LConn3
  _CN_128123911_220000_CN_128182735_220000/RConn1 -- T_128123911_220000_/LConn1 -- _CN_128123911_220000_CN_127255915_220000/LConn1
  _CN_128123911_220000_CN_128182735_220000/RConn2 -- T_128123911_220000_/LConn2 -- _CN_128123911_220000_CN_127255915_220000/LConn2
  _CN_128123911_220000_CN_128182735_220000/RConn3 -- T_128123911_220000_/LConn3 -- _CN_128123911_220000_CN_127255915_220000/LConn3 -- bus27/LConn1
  _CN_128123911_220000_CN_127255915_220000/RConn1 -- T_127255915_220000;66000_/LConn1 -- _CN_127261542_220000_CN_127255915_220000/LConn1 -- _CN_127243911_220000_CN_127255915_220000/LConn1 -- _CN_128125479_220000_CN_127255915_220000/LConn1
  _CN_128123911_220000_CN_127255915_220000/RConn2 -- T_127255915_220000;66000_/LConn2 -- _CN_127261542_220000_CN_127255915_220000/LConn2 -- _CN_127243911_220000_CN_127255915_220000/LConn2 -- _CN_128125479_220000_CN_127255915_220000/LConn2
  _CN_128123911_220000_CN_127255915_220000/RConn3 -- T_127255915_220000;66000_/LConn3 -- _CN_127261542_220000_CN_127255915_220000/LConn3 -- bus28/LConn1 -- _CN_127243911_220000_CN_127255915_220000/LConn3 -- _CN_128125479_220000_CN_127255915_220000/LConn3
  T_103998472_220000_/LConn1 -- _CN_103998472_220000_CN_126503845_220000/LConn1
  T_103998472_220000_/LConn2 -- _CN_103998472_220000_CN_126503845_220000/LConn2
  _CN_103998472_220000_CN_126503845_220000/LConn3 -- T_103998472_220000_/LConn3 -- bus29/LConn1
  T_126503845_220000;132000_/LConn1 -- _CN_103998472_220000_CN_126503845_220000/RConn1
  T_126503845_220000;132000_/LConn2 -- _CN_103998472_220000_CN_126503845_220000/RConn2
  _CN_103998472_220000_CN_126503845_220000/RConn3 -- T_126503845_220000;132000_/LConn3 -- bus30/LConn1
  T_213211662_220000_/LConn1 -- _CN_213211662_220000_CN_263290997_220000/RConn1
  T_213211662_220000_/LConn2 -- _CN_213211662_220000_CN_263290997_220000/RConn2
  _CN_213211662_220000_CN_263290997_220000/RConn3 -- T_213211662_220000_/LConn3 -- bus31/LConn1
  _CN_130229777_220000_CN_216227836_220000/LConn1 -- T_130229777_220000;66000_/LConn1 -- _CN_130229777_220000_CN_118310545_220000/LConn1
  _CN_130229777_220000_CN_216227836_220000/LConn2 -- T_130229777_220000;66000_/LConn2 -- _CN_130229777_220000_CN_118310545_220000/LConn2
  _CN_130229777_220000_CN_216227836_220000/LConn3 -- T_130229777_220000;66000_/LConn3 -- _CN_130229777_220000_CN_118310545_220000/LConn3 -- bus32/LConn1
  T_216227836_220000_/LConn1 -- _CN_130229777_220000_CN_216227836_220000/RConn1
  T_216227836_220000_/LConn2 -- _CN_130229777_220000_CN_216227836_220000/RConn2
  _CN_130229777_220000_CN_216227836_220000/RConn3 -- T_216227836_220000_/LConn3 -- bus33/LConn1
  _CN_130229777_220000_CN_118310545_220000/RConn1 -- T_118310545_500000;220000_/RConn1 -- _CN_97702932_220000_CN_118310545_220000/LConn1 -- L_118310545/LConn1
  _CN_130229777_220000_CN_118310545_220000/RConn2 -- T_118310545_500000;220000_/RConn2 -- _CN_97702932_220000_CN_118310545_220000/LConn2 -- L_118310545/LConn2
  _CN_130229777_220000_CN_118310545_220000/RConn3 -- T_118310545_500000;220000_/RConn3 -- _CN_97702932_220000_CN_118310545_220000/LConn3 -- L_118310545/LConn3 -- bus34/LConn1
  _CN_97702932_220000_CN_219687981_220000/LConn1 -- T_97702932_220000_/LConn1 -- _CN_97702932_220000_CN_92907650_220000/LConn1 -- _CN_97702932_220000_CN_130572646_220000/LConn1 -- _CN_97702932_220000_CN_118310545_220000/RConn1
  _CN_97702932_220000_CN_219687981_220000/LConn2 -- T_97702932_220000_/LConn2 -- _CN_97702932_220000_CN_92907650_220000/LConn2 -- _CN_97702932_220000_CN_130572646_220000/LConn2 -- _CN_97702932_220000_CN_118310545_220000/RConn2
  _CN_97702932_220000_CN_219687981_220000/LConn3 -- T_97702932_220000_/LConn3 -- _CN_97702932_220000_CN_92907650_220000/LConn3 -- _CN_97702932_220000_CN_130572646_220000/LConn3 -- bus35/LConn1 -- _CN_97702932_220000_CN_118310545_220000/RConn3
  _CN_97702932_220000_CN_219687981_220000/RConn1 -- T_219687981_220000_/LConn1 -- _CN_219687981_220000_CN_119907603_220000/LConn1
  _CN_97702932_220000_CN_219687981_220000/RConn2 -- T_219687981_220000_/LConn2 -- _CN_219687981_220000_CN_119907603_220000/LConn2
  _CN_97702932_220000_CN_219687981_220000/RConn3 -- T_219687981_220000_/LConn3 -- _CN_219687981_220000_CN_119907603_220000/LConn3 -- bus36/LConn1
  _CN_97702932_220000_CN_92907650_220000/RConn1 -- G_92907650_محطة_توليد_كهرباء_العين_السخنة/RConn1 -- _CN_130572646_220000_CN_92907650_220000/LConn1
  _CN_97702932_220000_CN_92907650_220000/RConn2 -- G_92907650_محطة_توليد_كهرباء_العين_السخنة/RConn2 -- _CN_130572646_220000_CN_92907650_220000/LConn2
  _CN_97702932_220000_CN_92907650_220000/RConn3 -- G_92907650_محطة_توليد_كهرباء_العين_السخنة/RConn3 -- _CN_130572646_220000_CN_92907650_220000/LConn3 -- bus37/LConn1
  _CN_97702932_220000_CN_130572646_220000/RConn1 -- T_130572646_220000_/LConn1 -- _CN_130572645_220000_CN_130572646_220000/LConn1 -- _CN_130572646_220000_CN_92907650_220000/RConn1
  _CN_97702932_220000_CN_130572646_220000/RConn2 -- T_130572646_220000_/LConn2 -- _CN_130572645_220000_CN_130572646_220000/LConn2 -- _CN_130572646_220000_CN_92907650_220000/RConn2
  _CN_97702932_220000_CN_130572646_220000/RConn3 -- T_130572646_220000_/LConn3 -- _CN_130572645_220000_CN_130572646_220000/LConn3 -- _CN_130572646_220000_CN_92907650_220000/RConn3 -- bus38/LConn1
  _CN_214809518_220000_CN_216093003_220000/LConn1 -- T_214809518_220000_/LConn1 -- _CN_214809518_220000_CN_276511906_220000/LConn1
  _CN_214809518_220000_CN_216093003_220000/LConn2 -- T_214809518_220000_/LConn2 -- _CN_214809518_220000_CN_276511906_220000/LConn2
  _CN_214809518_220000_CN_216093003_220000/LConn3 -- T_214809518_220000_/LConn3 -- _CN_214809518_220000_CN_276511906_220000/LConn3 -- bus39/LConn1
  _CN_214809518_220000_CN_216093003_220000/RConn1 -- T_216093003_220000_/LConn1 -- _CN_216214039_220000_CN_216093003_220000/LConn1
  _CN_214809518_220000_CN_216093003_220000/RConn2 -- T_216093003_220000_/LConn2 -- _CN_216214039_220000_CN_216093003_220000/LConn2
  _CN_214809518_220000_CN_216093003_220000/RConn3 -- T_216093003_220000_/LConn3 -- _CN_216214039_220000_CN_216093003_220000/LConn3 -- bus40/LConn1
  _CN_214809518_220000_CN_276511906_220000/RConn1 -- T_276511906_220000;66000_/LConn1 -- _CN_176719989_220000_CN_276511906_220000/LConn1
  _CN_214809518_220000_CN_276511906_220000/RConn2 -- T_276511906_220000;66000_/LConn2 -- _CN_176719989_220000_CN_276511906_220000/LConn2
  _CN_214809518_220000_CN_276511906_220000/RConn3 -- T_276511906_220000;66000_/LConn3 -- _CN_176719989_220000_CN_276511906_220000/LConn3 -- bus41/LConn1
  _CN_216214039_220000_CN_343022340_220000/LConn1 -- T_216214039_220000_/LConn1 -- _CN_216214039_220000_CN_216093003_220000/RConn1
  _CN_216214039_220000_CN_343022340_220000/LConn2 -- T_216214039_220000_/LConn2 -- _CN_216214039_220000_CN_216093003_220000/RConn2
  _CN_216214039_220000_CN_343022340_220000/LConn3 -- T_216214039_220000_/LConn3 -- _CN_216214039_220000_CN_216093003_220000/RConn3 -- bus42/LConn1
  _CN_216214039_220000_CN_343022340_220000/RConn1 -- T_343022340_220000_/LConn1 -- _CN_343022340_220000_CN_93699965_220000/LConn1
  _CN_216214039_220000_CN_343022340_220000/RConn2 -- T_343022340_220000_/LConn2 -- _CN_343022340_220000_CN_93699965_220000/LConn2
  _CN_216214039_220000_CN_343022340_220000/RConn3 -- T_343022340_220000_/LConn3 -- _CN_343022340_220000_CN_93699965_220000/LConn3 -- bus43/LConn1
  _CN_219020313_220000_CN_219032903_220000/LConn1 -- T_219020313_220000_/LConn1 -- _CN_219020313_220000_CN_95838096_220000/LConn1
  _CN_219020313_220000_CN_219032903_220000/LConn2 -- T_219020313_220000_/LConn2 -- _CN_219020313_220000_CN_95838096_220000/LConn2
  _CN_219020313_220000_CN_219032903_220000/LConn3 -- T_219020313_220000_/LConn3 -- _CN_219020313_220000_CN_95838096_220000/LConn3 -- bus44/LConn1
  _CN_219020313_220000_CN_219032903_220000/RConn1 -- T_219032903_220000_/LConn1 -- _CN_219032903_220000_CN_127398225_220000/LConn1
  _CN_219020313_220000_CN_219032903_220000/RConn2 -- T_219032903_220000_/LConn2 -- _CN_219032903_220000_CN_127398225_220000/LConn2
  _CN_219020313_220000_CN_219032903_220000/RConn3 -- T_219032903_220000_/LConn3 -- _CN_219032903_220000_CN_127398225_220000/LConn3 -- bus45/LConn1
  _CN_219020313_220000_CN_95838096_220000/RConn1 -- G_95838096_/RConn1 -- _CN_127243911_220000_CN_95838096_220000/LConn1 -- _CN_219005247_220000_CN_95838096_220000/LConn1
  _CN_219020313_220000_CN_95838096_220000/RConn2 -- G_95838096_/RConn2 -- _CN_127243911_220000_CN_95838096_220000/LConn2 -- _CN_219005247_220000_CN_95838096_220000/LConn2
  _CN_219020313_220000_CN_95838096_220000/RConn3 -- G_95838096_/RConn3 -- _CN_127243911_220000_CN_95838096_220000/LConn3 -- _CN_219005247_220000_CN_95838096_220000/LConn3 -- bus46/LConn1
  _CN_119907869_220000_CN_427608567_220000/LConn1 -- T_119907869_220000_/LConn1 -- _CN_119907869_220000_CN_119907603_220000/LConn1
  _CN_119907869_220000_CN_427608567_220000/LConn2 -- T_119907869_220000_/LConn2 -- _CN_119907869_220000_CN_119907603_220000/LConn2
  _CN_119907869_220000_CN_427608567_220000/LConn3 -- T_119907869_220000_/LConn3 -- _CN_119907869_220000_CN_119907603_220000/LConn3 -- bus47/LConn1
  T_427608567__/LConn1 -- _CN_119907869_220000_CN_427608567_220000/RConn1
  T_427608567__/LConn2 -- _CN_119907869_220000_CN_427608567_220000/RConn2
  _CN_119907869_220000_CN_427608567_220000/RConn3 -- T_427608567__/LConn3 -- bus48/LConn1
  _CN_119907869_220000_CN_119907603_220000/RConn1 -- T_119907603_220000_/LConn1 -- _CN_219687981_220000_CN_119907603_220000/RConn1 -- _CN_92878367_220000_CN_119907603_220000/LConn1
  _CN_119907869_220000_CN_119907603_220000/RConn2 -- T_119907603_220000_/LConn2 -- _CN_219687981_220000_CN_119907603_220000/RConn2 -- _CN_92878367_220000_CN_119907603_220000/LConn2
  _CN_119907869_220000_CN_119907603_220000/RConn3 -- T_119907603_220000_/LConn3 -- _CN_219687981_220000_CN_119907603_220000/RConn3 -- bus49/LConn1 -- _CN_92878367_220000_CN_119907603_220000/LConn3
  _CN_92878367_220000_CN_105191630_220000/LConn1 -- T_92878367_220000_/LConn1 -- _CN_92878367_220000_CN_119909663_220000/LConn1 -- _CN_92878367_220000_CN_119907603_220000/RConn1 -- _CN_92878367_220000_CN_90608610_220000/LConn1
  _CN_92878367_220000_CN_105191630_220000/LConn2 -- T_92878367_220000_/LConn2 -- _CN_92878367_220000_CN_119909663_220000/LConn2 -- _CN_92878367_220000_CN_119907603_220000/RConn2 -- _CN_92878367_220000_CN_90608610_220000/LConn2
  _CN_92878367_220000_CN_105191630_220000/LConn3 -- T_92878367_220000_/LConn3 -- _CN_92878367_220000_CN_119909663_220000/LConn3 -- _CN_92878367_220000_CN_119907603_220000/RConn3 -- _CN_92878367_220000_CN_90608610_220000/LConn3 -- bus50/LConn1
  _CN_92878367_220000_CN_105191630_220000/RConn1 -- T_105191630_220000;66000_/LConn1 -- _CN_102988963_220000_CN_105191630_220000/LConn1 -- _CN_105191630_220000_CN_427790093_220000/LConn1 -- _CN_105191630_220000_CN_90608610_220000/LConn1
  _CN_92878367_220000_CN_105191630_220000/RConn2 -- T_105191630_220000;66000_/LConn2 -- _CN_102988963_220000_CN_105191630_220000/LConn2 -- _CN_105191630_220000_CN_427790093_220000/LConn2 -- _CN_105191630_220000_CN_90608610_220000/LConn2
  _CN_92878367_220000_CN_105191630_220000/RConn3 -- T_105191630_220000;66000_/LConn3 -- _CN_102988963_220000_CN_105191630_220000/LConn3 -- _CN_105191630_220000_CN_427790093_220000/LConn3 -- _CN_105191630_220000_CN_90608610_220000/LConn3 -- bus51/LConn1
  T_119909663_220000_/LConn1 -- _CN_92878367_220000_CN_119909663_220000/RConn1
  T_119909663_220000_/LConn2 -- _CN_92878367_220000_CN_119909663_220000/RConn2
  _CN_92878367_220000_CN_119909663_220000/RConn3 -- T_119909663_220000_/LConn3 -- bus52/LConn1
  _CN_92878367_220000_CN_90608610_220000/RConn1 -- T_90608610_220000_/RConn1 -- _CN_105191630_220000_CN_90608610_220000/RConn1 -- _CN_90608610_220000_CN_105569177_220000/LConn1 -- L_90608610/LConn1
  _CN_92878367_220000_CN_90608610_220000/RConn2 -- T_90608610_220000_/RConn2 -- _CN_105191630_220000_CN_90608610_220000/RConn2 -- _CN_90608610_220000_CN_105569177_220000/LConn2 -- L_90608610/LConn2
  _CN_92878367_220000_CN_90608610_220000/RConn3 -- T_90608610_220000_/RConn3 -- _CN_105191630_220000_CN_90608610_220000/RConn3 -- _CN_90608610_220000_CN_105569177_220000/LConn3 -- L_90608610/LConn3 -- bus53/LConn1
  _CN_98663458_220000_CN_98663507_220000/LConn1 -- T_98663458_220000;66000_/LConn1 -- _CN_98663458_220000_CN_118301256_220000/LConn1
  _CN_98663458_220000_CN_98663507_220000/LConn2 -- T_98663458_220000;66000_/LConn2 -- _CN_98663458_220000_CN_118301256_220000/LConn2
  _CN_98663458_220000_CN_98663507_220000/LConn3 -- T_98663458_220000;66000_/LConn3 -- _CN_98663458_220000_CN_118301256_220000/LConn3 -- bus54/LConn1
  _CN_98663458_220000_CN_98663507_220000/RConn1 -- T_98663507_220000;66000_/LConn1 -- _CN_98663507_220000_CN_117671808_220000/LConn1
  _CN_98663458_220000_CN_98663507_220000/RConn2 -- T_98663507_220000;66000_/LConn2 -- _CN_98663507_220000_CN_117671808_220000/LConn2
  _CN_98663458_220000_CN_98663507_220000/RConn3 -- T_98663507_220000;66000_/LConn3 -- _CN_98663507_220000_CN_117671808_220000/LConn3 -- bus55/LConn1
  _CN_98663458_220000_CN_118301256_220000/RConn1 -- G_118301256_/RConn1 -- _CN_426156916_220000_CN_118301256_220000/LConn1 -- _CN_119584035_220000_CN_118301256_220000/LConn1 -- _CN_426156915_220000_CN_118301256_220000/LConn1 -- _CN_118310545_500000_CN_118301256_220000/LConn1
  _CN_98663458_220000_CN_118301256_220000/RConn2 -- G_118301256_/RConn2 -- _CN_426156916_220000_CN_118301256_220000/LConn2 -- _CN_119584035_220000_CN_118301256_220000/LConn2 -- _CN_426156915_220000_CN_118301256_220000/LConn2 -- _CN_118310545_500000_CN_118301256_220000/LConn2
  _CN_98663458_220000_CN_118301256_220000/RConn3 -- G_118301256_/RConn3 -- _CN_426156916_220000_CN_118301256_220000/LConn3 -- _CN_119584035_220000_CN_118301256_220000/LConn3 -- _CN_426156915_220000_CN_118301256_220000/LConn3 -- _CN_118310545_500000_CN_118301256_220000/LConn3 -- bus56/LConn1
  _CN_128125479_220000_CN_128129616_220000/LConn1 -- T_128125479_220000_/LConn1 -- _CN_128125479_220000_CN_127255915_220000/RConn1
  _CN_128125479_220000_CN_128129616_220000/LConn2 -- T_128125479_220000_/LConn2 -- _CN_128125479_220000_CN_127255915_220000/RConn2
  _CN_128125479_220000_CN_128129616_220000/LConn3 -- T_128125479_220000_/LConn3 -- _CN_128125479_220000_CN_127255915_220000/RConn3 -- bus57/LConn1
  _CN_128125479_220000_CN_128129616_220000/RConn1 -- T_128129616_220000_/LConn1 -- _CN_128129616_220000_CN_128182735_220000/RConn1 -- _CN_128129616_220000_CN_128205604_220000/LConn1
  _CN_128125479_220000_CN_128129616_220000/RConn2 -- T_128129616_220000_/LConn2 -- _CN_128129616_220000_CN_128182735_220000/RConn2 -- _CN_128129616_220000_CN_128205604_220000/LConn2
  _CN_128125479_220000_CN_128129616_220000/RConn3 -- T_128129616_220000_/LConn3 -- _CN_128129616_220000_CN_128182735_220000/RConn3 -- _CN_128129616_220000_CN_128205604_220000/LConn3 -- bus58/LConn1
  _CN_130435119_220000_CN_219583071_220000/RConn1 -- T_219583071_220000;66000_/LConn1 -- _CN_219583071_220000_CN_426825830_220000/LConn1
  _CN_130435119_220000_CN_219583071_220000/RConn2 -- T_219583071_220000;66000_/LConn2 -- _CN_219583071_220000_CN_426825830_220000/LConn2
  _CN_130435119_220000_CN_219583071_220000/RConn3 -- T_219583071_220000;66000_/LConn3 -- _CN_219583071_220000_CN_426825830_220000/LConn3 -- bus59/LConn1
  T_219295621_220000_/LConn1 -- _CN_130435119_220000_CN_219295621_220000/RConn1
  T_219295621_220000_/LConn2 -- _CN_130435119_220000_CN_219295621_220000/RConn2
  _CN_130435119_220000_CN_219295621_220000/RConn3 -- T_219295621_220000_/LConn3 -- bus60/LConn1
  _CN_426596409_220000_CN_115491527_220000/LConn1 -- T_426596409_220000_/LConn1 -- _CN_426596409_220000_CN_117342821_220000/LConn1
  _CN_426596409_220000_CN_115491527_220000/LConn2 -- T_426596409_220000_/LConn2 -- _CN_426596409_220000_CN_117342821_220000/LConn2
  _CN_426596409_220000_CN_115491527_220000/LConn3 -- T_426596409_220000_/LConn3 -- _CN_426596409_220000_CN_117342821_220000/LConn3 -- bus61/LConn1
  _CN_426596409_220000_CN_115491527_220000/RConn1 -- T_115491527_500000;220000;132000_/RConn1 -- _CN_115491527_220000_CN_130524402_220000/LConn1 -- _CN_115491527_220000_CN_213203948_220000/LConn1 -- _CN_115491527_220000_CN_115498840_220000/LConn1
  _CN_426596409_220000_CN_115491527_220000/RConn2 -- T_115491527_500000;220000;132000_/RConn2 -- _CN_115491527_220000_CN_130524402_220000/LConn2 -- _CN_115491527_220000_CN_213203948_220000/LConn2 -- _CN_115491527_220000_CN_115498840_220000/LConn2
  _CN_426596409_220000_CN_115491527_220000/RConn3 -- T_115491527_500000;220000;132000_/RConn3 -- _CN_115491527_220000_CN_130524402_220000/LConn3 -- bus62/LConn1 -- _CN_115491527_220000_CN_213203948_220000/LConn3 -- _CN_115491527_220000_CN_115498840_220000/LConn3
  _CN_426596409_220000_CN_117342821_220000/RConn1 -- T_117342821_220000_/LConn1 -- _CN_117342821_220000_CN_117381489_220000/LConn1
  _CN_426596409_220000_CN_117342821_220000/RConn2 -- T_117342821_220000_/LConn2 -- _CN_117342821_220000_CN_117381489_220000/LConn2
  _CN_426596409_220000_CN_117342821_220000/RConn3 -- T_117342821_220000_/LConn3 -- _CN_117342821_220000_CN_117381489_220000/LConn3 -- bus63/LConn1
  _CN_219583071_220000_CN_426825830_220000/RConn1 -- T_426825830_220000_/LConn1 -- _CN_426825830_220000_CN_213203948_220000/LConn1
  _CN_219583071_220000_CN_426825830_220000/RConn2 -- T_426825830_220000_/LConn2 -- _CN_426825830_220000_CN_213203948_220000/LConn2
  _CN_219583071_220000_CN_426825830_220000/RConn3 -- T_426825830_220000_/LConn3 -- _CN_426825830_220000_CN_213203948_220000/LConn3 -- bus64/LConn1
  _CN_120521277_220000_CN_120516781_220000/LConn1 -- T_120521277__/LConn1 -- _CN_120521277_220000_CN_123223445_220000/LConn1 -- _CN_120521277_220000_CN_122132699_220000/LConn1
  _CN_120521277_220000_CN_120516781_220000/LConn2 -- T_120521277__/LConn2 -- _CN_120521277_220000_CN_123223445_220000/LConn2 -- _CN_120521277_220000_CN_122132699_220000/LConn2
  _CN_120521277_220000_CN_120516781_220000/LConn3 -- T_120521277__/LConn3 -- _CN_120521277_220000_CN_123223445_220000/LConn3 -- _CN_120521277_220000_CN_122132699_220000/LConn3 -- bus65/LConn1
  T_120516781__/LConn1 -- _CN_120521277_220000_CN_120516781_220000/RConn1
  T_120516781__/LConn2 -- _CN_120521277_220000_CN_120516781_220000/RConn2
  _CN_120521277_220000_CN_120516781_220000/RConn3 -- T_120516781__/LConn3 -- bus66/LConn1
  _CN_120521277_220000_CN_123223445_220000/RConn1 -- T_123223445_220000;66000_/LConn1 -- _CN_122238112_220000_CN_123223445_220000/LConn1 -- _CN_123466581_220000_CN_123223445_220000/LConn1 -- _CN_123223445_220000_CN_105694639_220000/LConn1
  _CN_120521277_220000_CN_123223445_220000/RConn2 -- T_123223445_220000;66000_/LConn2 -- _CN_122238112_220000_CN_123223445_220000/LConn2 -- _CN_123466581_220000_CN_123223445_220000/LConn2 -- _CN_123223445_220000_CN_105694639_220000/LConn2
  _CN_120521277_220000_CN_123223445_220000/RConn3 -- T_123223445_220000;66000_/LConn3 -- _CN_122238112_220000_CN_123223445_220000/LConn3 -- _CN_123466581_220000_CN_123223445_220000/LConn3 -- _CN_123223445_220000_CN_105694639_220000/LConn3 -- bus67/LConn1
  _CN_120521277_220000_CN_122132699_220000/RConn1 -- T_122132699_220000;66000_/LConn1 -- _CN_122132699_220000_CN_127212017_220000/LConn1 -- _CN_122238112_220000_CN_122132699_220000/LConn1
  _CN_120521277_220000_CN_122132699_220000/RConn2 -- T_122132699_220000;66000_/LConn2 -- _CN_122132699_220000_CN_127212017_220000/LConn2 -- _CN_122238112_220000_CN_122132699_220000/LConn2
  _CN_120521277_220000_CN_122132699_220000/RConn3 -- T_122132699_220000;66000_/LConn3 -- _CN_122132699_220000_CN_127212017_220000/LConn3 -- bus68/LConn1 -- _CN_122238112_220000_CN_122132699_220000/LConn3
  T_117528642_220000;66000_/LConn1 -- _CN_117528642_220000_CN_93583051_220000/LConn1
  T_117528642_220000;66000_/LConn2 -- _CN_117528642_220000_CN_93583051_220000/LConn2
  _CN_117528642_220000_CN_93583051_220000/LConn3 -- T_117528642_220000;66000_/LConn3 -- bus69/LConn1
  _CN_117528642_220000_CN_93583051_220000/RConn1 -- G_93583051_Asyut_refinery/RConn1 -- _CN_117393191_220000_CN_93583051_220000/LConn1
  _CN_117528642_220000_CN_93583051_220000/RConn2 -- G_93583051_Asyut_refinery/RConn2 -- _CN_117393191_220000_CN_93583051_220000/LConn2
  _CN_117528642_220000_CN_93583051_220000/RConn3 -- G_93583051_Asyut_refinery/RConn3 -- _CN_117393191_220000_CN_93583051_220000/LConn3 -- bus70/LConn1
  T_218898508_220000;66000_/LConn1 -- _CN_218898508_220000_CN_93650324_220000/RConn1
  T_218898508_220000;66000_/LConn2 -- _CN_218898508_220000_CN_93650324_220000/RConn2
  _CN_218898508_220000_CN_93650324_220000/RConn3 -- T_218898508_220000;66000_/LConn3 -- bus71/LConn1
  _CN_128129616_220000_CN_128205604_220000/RConn1 -- T_128205604_500000_/RConn1 -- _CN_128205604_220000_CN_28830169_220000/LConn1 -- L_128205604/LConn1
  _CN_128129616_220000_CN_128205604_220000/RConn2 -- T_128205604_500000_/RConn2 -- _CN_128205604_220000_CN_28830169_220000/LConn2 -- L_128205604/LConn2
  _CN_128129616_220000_CN_128205604_220000/RConn3 -- T_128205604_500000_/RConn3 -- _CN_128205604_220000_CN_28830169_220000/LConn3 -- L_128205604/LConn3 -- bus72/LConn1
  _CN_126280786_220000_CN_131236227_220000/LConn1 -- T_126280786_220000;66000_/LConn1 -- _CN_126280786_220000_CN_265751903_220000/LConn1 -- _CN_126280786_220000_CN_126200917_220000/LConn1
  _CN_126280786_220000_CN_131236227_220000/LConn2 -- T_126280786_220000;66000_/LConn2 -- _CN_126280786_220000_CN_265751903_220000/LConn2 -- _CN_126280786_220000_CN_126200917_220000/LConn2
  _CN_126280786_220000_CN_131236227_220000/LConn3 -- T_126280786_220000;66000_/LConn3 -- _CN_126280786_220000_CN_265751903_220000/LConn3 -- _CN_126280786_220000_CN_126200917_220000/LConn3 -- bus73/LConn1
  _CN_126280786_220000_CN_131236227_220000/RConn1 -- G_131236227_El_Mex_refinery/RConn1 -- _CN_131239138_220000_CN_131236227_220000/LConn1 -- _CN_218972674_500000_CN_131236227_220000/LConn1
  _CN_126280786_220000_CN_131236227_220000/RConn2 -- G_131236227_El_Mex_refinery/RConn2 -- _CN_131239138_220000_CN_131236227_220000/LConn2 -- _CN_218972674_500000_CN_131236227_220000/LConn2
  _CN_126280786_220000_CN_131236227_220000/RConn3 -- G_131236227_El_Mex_refinery/RConn3 -- _CN_131239138_220000_CN_131236227_220000/LConn3 -- _CN_218972674_500000_CN_131236227_220000/LConn3 -- bus74/LConn1
  T_265751903__/LConn1 -- _CN_126280786_220000_CN_265751903_220000/RConn1
  T_265751903__/LConn2 -- _CN_126280786_220000_CN_265751903_220000/RConn2
  _CN_126280786_220000_CN_265751903_220000/RConn3 -- T_265751903__/LConn3 -- bus75/LConn1
  T_126200917_220000_/LConn1 -- _CN_126280786_220000_CN_126200917_220000/RConn1
  T_126200917_220000_/LConn2 -- _CN_126280786_220000_CN_126200917_220000/RConn2
  _CN_126280786_220000_CN_126200917_220000/RConn3 -- T_126200917_220000_/LConn3 -- bus76/LConn1
  T_117671808_220000_/LConn1 -- _CN_98663507_220000_CN_117671808_220000/RConn1
  T_117671808_220000_/LConn2 -- _CN_98663507_220000_CN_117671808_220000/RConn2
  _CN_98663507_220000_CN_117671808_220000/RConn3 -- T_117671808_220000_/LConn3 -- bus77/LConn1
  T_218975834_220000_/LConn1 -- _CN_218975834_220000_CN_218976990_220000/LConn1
  T_218975834_220000_/LConn2 -- _CN_218975834_220000_CN_218976990_220000/LConn2
  _CN_218975834_220000_CN_218976990_220000/LConn3 -- T_218975834_220000_/LConn3 -- bus78/LConn1
  _CN_218975834_220000_CN_218976990_220000/RConn1 -- T_218976990_220000_/LConn1 -- _CN_218980895_220000_CN_218976990_220000/LConn1
  _CN_218975834_220000_CN_218976990_220000/RConn2 -- T_218976990_220000_/LConn2 -- _CN_218980895_220000_CN_218976990_220000/LConn2
  _CN_218975834_220000_CN_218976990_220000/RConn3 -- T_218976990_220000_/LConn3 -- _CN_218980895_220000_CN_218976990_220000/LConn3 -- bus79/LConn1
  _CN_216224349_220000_CN_130572645_220000/LConn1 -- T_216224349__Zafarana_7/LConn1 -- _CN_216224349_220000_CN_427596550_220000/LConn1
  _CN_216224349_220000_CN_130572645_220000/LConn2 -- T_216224349__Zafarana_7/LConn2 -- _CN_216224349_220000_CN_427596550_220000/LConn2
  _CN_216224349_220000_CN_130572645_220000/LConn3 -- T_216224349__Zafarana_7/LConn3 -- _CN_216224349_220000_CN_427596550_220000/LConn3 -- bus80/LConn1
  _CN_216224349_220000_CN_130572645_220000/RConn1 -- T_130572645__Zafarana_7/LConn1 -- _CN_130572645_220000_CN_130572646_220000/RConn1
  _CN_216224349_220000_CN_130572645_220000/RConn2 -- T_130572645__Zafarana_7/LConn2 -- _CN_130572645_220000_CN_130572646_220000/RConn2
  _CN_216224349_220000_CN_130572645_220000/RConn3 -- T_130572645__Zafarana_7/LConn3 -- _CN_130572645_220000_CN_130572646_220000/RConn3 -- bus81/LConn1
  T_427596550__El_Zayt_wind_farm/LConn1 -- _CN_216224349_220000_CN_427596550_220000/RConn1
  T_427596550__El_Zayt_wind_farm/LConn2 -- _CN_216224349_220000_CN_427596550_220000/RConn2
  _CN_216224349_220000_CN_427596550_220000/RConn3 -- T_427596550__El_Zayt_wind_farm/LConn3 -- bus82/LConn1
  _CN_103010149_220000_CN_103015033_220000/LConn1 -- T_103010149_500000_/RConn1 -- L_103010149/LConn1
  _CN_103010149_220000_CN_103015033_220000/LConn2 -- T_103010149_500000_/RConn2 -- L_103010149/LConn2
  _CN_103010149_220000_CN_103015033_220000/LConn3 -- T_103010149_500000_/RConn3 -- L_103010149/LConn3 -- bus83/LConn1
  _CN_103010149_220000_CN_103015033_220000/RConn1 -- T_103015033_220000;66000_/LConn1 -- _CN_103015033_220000_CN_123466581_220000/LConn1
  _CN_103010149_220000_CN_103015033_220000/RConn2 -- T_103015033_220000;66000_/LConn2 -- _CN_103015033_220000_CN_123466581_220000/LConn2
  _CN_103010149_220000_CN_103015033_220000/RConn3 -- T_103015033_220000;66000_/LConn3 -- _CN_103015033_220000_CN_123466581_220000/LConn3 -- bus84/LConn1
  _CN_117342821_220000_CN_117381489_220000/RConn1 -- T_117381489_220000;66000_/LConn1 -- _CN_117381489_220000_CN_426347972_220000/LConn1
  _CN_117342821_220000_CN_117381489_220000/RConn2 -- T_117381489_220000;66000_/LConn2 -- _CN_117381489_220000_CN_426347972_220000/LConn2
  _CN_117342821_220000_CN_117381489_220000/RConn3 -- T_117381489_220000;66000_/LConn3 -- _CN_117381489_220000_CN_426347972_220000/LConn3 -- bus85/LConn1
  _CN_426825830_220000_CN_213203948_220000/RConn1 -- T_213203948_220000;132000;66000_/LConn1 -- _CN_99788079_220000_CN_213203948_220000/LConn1 -- _CN_115491527_220000_CN_213203948_220000/RConn1
  _CN_426825830_220000_CN_213203948_220000/RConn2 -- T_213203948_220000;132000;66000_/LConn2 -- _CN_99788079_220000_CN_213203948_220000/LConn2 -- _CN_115491527_220000_CN_213203948_220000/RConn2
  _CN_426825830_220000_CN_213203948_220000/RConn3 -- T_213203948_220000;132000;66000_/LConn3 -- _CN_99788079_220000_CN_213203948_220000/LConn3 -- bus86/LConn1 -- _CN_115491527_220000_CN_213203948_220000/RConn3
  _CN_97721447_220000_CN_97721460_220000/LConn1 -- T_97721447_220000;66000_/LConn1 -- _CN_97721447_220000_CN_176719989_220000/LConn1
  _CN_97721447_220000_CN_97721460_220000/LConn2 -- T_97721447_220000;66000_/LConn2 -- _CN_97721447_220000_CN_176719989_220000/LConn2
  _CN_97721447_220000_CN_97721460_220000/LConn3 -- T_97721447_220000;66000_/LConn3 -- _CN_97721447_220000_CN_176719989_220000/LConn3 -- bus87/LConn1
  _CN_97721447_220000_CN_97721460_220000/RConn1 -- T_97721460_220000_/RConn1 -- L_97721460/LConn1
  _CN_97721447_220000_CN_97721460_220000/RConn2 -- T_97721460_220000_/RConn2 -- L_97721460/LConn2
  _CN_97721447_220000_CN_97721460_220000/RConn3 -- T_97721460_220000_/RConn3 -- L_97721460/LConn3 -- bus88/LConn1
  _CN_97721447_220000_CN_176719989_220000/RConn1 -- T_176719989_220000;66000_/LConn1 -- _CN_176719989_220000_CN_276511906_220000/RConn1
  _CN_97721447_220000_CN_176719989_220000/RConn2 -- T_176719989_220000;66000_/LConn2 -- _CN_176719989_220000_CN_276511906_220000/RConn2
  _CN_97721447_220000_CN_176719989_220000/RConn3 -- T_176719989_220000;66000_/LConn3 -- _CN_176719989_220000_CN_276511906_220000/RConn3 -- bus89/LConn1
  T_93714538_220000_/LConn1 -- _CN_93714538_220000_CN_105694639_220000/LConn1
  T_93714538_220000_/LConn2 -- _CN_93714538_220000_CN_105694639_220000/LConn2
  _CN_93714538_220000_CN_105694639_220000/LConn3 -- T_93714538_220000_/LConn3 -- bus90/LConn1
  _CN_93714538_220000_CN_105694639_220000/RConn1 -- T_105694639_220000_/LConn1 -- _CN_123223445_220000_CN_105694639_220000/RConn1 -- _CN_105694639_220000_CN_105569177_220000/LConn1
  _CN_93714538_220000_CN_105694639_220000/RConn2 -- T_105694639_220000_/LConn2 -- _CN_123223445_220000_CN_105694639_220000/RConn2 -- _CN_105694639_220000_CN_105569177_220000/LConn2
  _CN_93714538_220000_CN_105694639_220000/RConn3 -- T_105694639_220000_/LConn3 -- _CN_123223445_220000_CN_105694639_220000/RConn3 -- _CN_105694639_220000_CN_105569177_220000/LConn3 -- bus91/LConn1
  _CN_103015033_220000_CN_123466581_220000/RConn1 -- T_123466581_220000;66000_/LConn1 -- _CN_123466581_220000_CN_105569177_220000/LConn1 -- _CN_123466581_220000_CN_123223445_220000/RConn1
  _CN_103015033_220000_CN_123466581_220000/RConn2 -- T_123466581_220000;66000_/LConn2 -- _CN_123466581_220000_CN_105569177_220000/LConn2 -- _CN_123466581_220000_CN_123223445_220000/RConn2
  _CN_103015033_220000_CN_123466581_220000/RConn3 -- T_123466581_220000;66000_/LConn3 -- _CN_123466581_220000_CN_105569177_220000/LConn3 -- _CN_123466581_220000_CN_123223445_220000/RConn3 -- bus92/LConn1
  _CN_127243911_220000_CN_95838096_220000/RConn1 -- T_127243911_220000;66000_/LConn1 -- _CN_127243911_220000_CN_127212017_220000/LConn1 -- _CN_127243911_220000_CN_127255915_220000/RConn1
  _CN_127243911_220000_CN_95838096_220000/RConn2 -- T_127243911_220000;66000_/LConn2 -- _CN_127243911_220000_CN_127212017_220000/LConn2 -- _CN_127243911_220000_CN_127255915_220000/RConn2
  _CN_127243911_220000_CN_95838096_220000/RConn3 -- T_127243911_220000;66000_/LConn3 -- _CN_127243911_220000_CN_127212017_220000/LConn3 -- bus93/LConn1 -- _CN_127243911_220000_CN_127255915_220000/RConn3
  _CN_127243911_220000_CN_127212017_220000/RConn1 -- G_127212017_Damietta/RConn1 -- _CN_122132699_220000_CN_127212017_220000/RConn1 -- _CN_122238112_220000_CN_127212017_220000/LConn1
  _CN_127243911_220000_CN_127212017_220000/RConn2 -- G_127212017_Damietta/RConn2 -- _CN_122132699_220000_CN_127212017_220000/RConn2 -- _CN_122238112_220000_CN_127212017_220000/LConn2
  _CN_127243911_220000_CN_127212017_220000/RConn3 -- G_127212017_Damietta/RConn3 -- _CN_122132699_220000_CN_127212017_220000/RConn3 -- bus94/LConn1 -- _CN_122238112_220000_CN_127212017_220000/LConn3
  _CN_97852047_220000_CN_118345956_220000/LConn1 -- T_97852047_220000_/LConn1 -- _CN_97852047_220000_CN_419686238_220000/LConn1
  _CN_97852047_220000_CN_118345956_220000/LConn2 -- T_97852047_220000_/LConn2 -- _CN_97852047_220000_CN_419686238_220000/LConn2
  _CN_97852047_220000_CN_118345956_220000/LConn3 -- T_97852047_220000_/LConn3 -- _CN_97852047_220000_CN_419686238_220000/LConn3 -- bus95/LConn1
  _CN_97852047_220000_CN_118345956_220000/RConn1 -- T_118345956_220000_/LConn1 -- _CN_118345956_220000_CN_94566888_220000/LConn1
  _CN_97852047_220000_CN_118345956_220000/RConn2 -- T_118345956_220000_/LConn2 -- _CN_118345956_220000_CN_94566888_220000/LConn2
  _CN_97852047_220000_CN_118345956_220000/RConn3 -- T_118345956_220000_/LConn3 -- _CN_118345956_220000_CN_94566888_220000/LConn3 -- bus96/LConn1
  T_419686238__/LConn1 -- _CN_97852047_220000_CN_419686238_220000/RConn1
  T_419686238__/LConn2 -- _CN_97852047_220000_CN_419686238_220000/RConn2
  _CN_97852047_220000_CN_419686238_220000/RConn3 -- T_419686238__/LConn3 -- bus97/LConn1
  T_102988954_220000_/LConn1 -- _CN_102988954_220000_CN_102988963_220000/LConn1
  T_102988954_220000_/LConn2 -- _CN_102988954_220000_CN_102988963_220000/LConn2
  _CN_102988954_220000_CN_102988963_220000/LConn3 -- T_102988954_220000_/LConn3 -- bus98/LConn1
  _CN_102988954_220000_CN_102988963_220000/RConn1 -- T_102988963_220000_/LConn1 -- _CN_102988963_220000_CN_105191630_220000/RConn1
  _CN_102988954_220000_CN_102988963_220000/RConn2 -- T_102988963_220000_/LConn2 -- _CN_102988963_220000_CN_105191630_220000/RConn2
  _CN_102988954_220000_CN_102988963_220000/RConn3 -- T_102988963_220000_/LConn3 -- _CN_102988963_220000_CN_105191630_220000/RConn3 -- bus99/LConn1
  _CN_122238112_220000_CN_122132699_220000/RConn1 -- T_122238112_220000;66000_/LConn1 -- _CN_122238112_220000_CN_127212017_220000/RConn1 -- _CN_122238112_220000_CN_123223445_220000/RConn1
  _CN_122238112_220000_CN_122132699_220000/RConn2 -- T_122238112_220000;66000_/LConn2 -- _CN_122238112_220000_CN_127212017_220000/RConn2 -- _CN_122238112_220000_CN_123223445_220000/RConn2
  _CN_122238112_220000_CN_122132699_220000/RConn3 -- T_122238112_220000;66000_/LConn3 -- _CN_122238112_220000_CN_127212017_220000/RConn3 -- _CN_122238112_220000_CN_123223445_220000/RConn3 -- bus100/LConn1
  T_120516782_220000_/LConn1 -- _CN_120516782_220000_CN_93699965_220000/LConn1
  T_120516782_220000_/LConn2 -- _CN_120516782_220000_CN_93699965_220000/LConn2
  _CN_120516782_220000_CN_93699965_220000/LConn3 -- T_120516782_220000_/LConn3 -- bus101/LConn1
  _CN_120516782_220000_CN_93699965_220000/RConn1 -- T_93699965_220000;66000_/LConn1 -- _CN_93699965_220000_CN_93650324_220000/RConn1 -- _CN_343022340_220000_CN_93699965_220000/RConn1
  _CN_120516782_220000_CN_93699965_220000/RConn2 -- T_93699965_220000;66000_/LConn2 -- _CN_93699965_220000_CN_93650324_220000/RConn2 -- _CN_343022340_220000_CN_93699965_220000/RConn2
  _CN_120516782_220000_CN_93699965_220000/RConn3 -- T_93699965_220000;66000_/LConn3 -- _CN_93699965_220000_CN_93650324_220000/RConn3 -- bus102/LConn1 -- _CN_343022340_220000_CN_93699965_220000/RConn3
  _CN_426156916_220000_CN_94566888_220000/LConn1 -- T_426156916__/LConn1 -- _CN_426156916_220000_CN_118301256_220000/RConn1
  _CN_426156916_220000_CN_94566888_220000/LConn2 -- T_426156916__/LConn2 -- _CN_426156916_220000_CN_118301256_220000/RConn2
  _CN_426156916_220000_CN_94566888_220000/LConn3 -- T_426156916__/LConn3 -- _CN_426156916_220000_CN_118301256_220000/RConn3 -- bus103/LConn1
  _CN_426156916_220000_CN_94566888_220000/RConn1 -- T_94566888_220000;66000_/LConn1 -- _CN_118345956_220000_CN_94566888_220000/RConn1 -- _CN_99494604_220000_CN_94566888_220000/LConn1
  _CN_426156916_220000_CN_94566888_220000/RConn2 -- T_94566888_220000;66000_/LConn2 -- _CN_118345956_220000_CN_94566888_220000/RConn2 -- _CN_99494604_220000_CN_94566888_220000/LConn2
  _CN_426156916_220000_CN_94566888_220000/RConn3 -- T_94566888_220000;66000_/LConn3 -- _CN_118345956_220000_CN_94566888_220000/RConn3 -- bus104/LConn1 -- _CN_99494604_220000_CN_94566888_220000/LConn3
  _CN_218980895_220000_CN_218976990_220000/RConn1 -- T_218980895_220000_/LConn1 -- _CN_218980895_220000_CN_218983235_220000/LConn1
  _CN_218980895_220000_CN_218976990_220000/RConn2 -- T_218980895_220000_/LConn2 -- _CN_218980895_220000_CN_218983235_220000/LConn2
  _CN_218980895_220000_CN_218976990_220000/RConn3 -- T_218980895_220000_/LConn3 -- _CN_218980895_220000_CN_218983235_220000/LConn3 -- bus105/LConn1
  T_218983235_220000_/LConn1 -- _CN_218980895_220000_CN_218983235_220000/RConn1
  T_218983235_220000_/LConn2 -- _CN_218980895_220000_CN_218983235_220000/RConn2
  _CN_218980895_220000_CN_218983235_220000/RConn3 -- T_218983235_220000_/LConn3 -- bus106/LConn1
  T_263365083__/LConn1 -- _CN_263290997_220000_CN_263365083_220000/RConn1
  T_263365083__/LConn2 -- _CN_263290997_220000_CN_263365083_220000/RConn2
  _CN_263290997_220000_CN_263365083_220000/RConn3 -- T_263365083__/LConn3 -- bus107/LConn1
  T_115498840__/LConn1 -- _CN_115491527_220000_CN_115498840_220000/RConn1
  T_115498840__/LConn2 -- _CN_115491527_220000_CN_115498840_220000/RConn2
  _CN_115491527_220000_CN_115498840_220000/RConn3 -- T_115498840__/LConn3 -- bus108/LConn1
  T_130524402_220000_/LConn1 -- _CN_115491527_220000_CN_130524402_220000/RConn1
  T_130524402_220000_/LConn2 -- _CN_115491527_220000_CN_130524402_220000/RConn2
  _CN_115491527_220000_CN_130524402_220000/RConn3 -- T_130524402_220000_/LConn3 -- bus109/LConn1
  T_99494604_220000_/LConn1 -- _CN_99494604_220000_CN_94566888_220000/RConn1
  T_99494604_220000_/LConn2 -- _CN_99494604_220000_CN_94566888_220000/RConn2
  _CN_99494604_220000_CN_94566888_220000/RConn3 -- T_99494604_220000_/LConn3 -- bus110/LConn1
  T_427790093__/LConn1 -- _CN_105191630_220000_CN_427790093_220000/RConn1
  T_427790093__/LConn2 -- _CN_105191630_220000_CN_427790093_220000/RConn2
  _CN_105191630_220000_CN_427790093_220000/RConn3 -- T_427790093__/LConn3 -- bus111/LConn1
  _CN_127261542_220000_CN_127255915_220000/RConn1 -- T_127261542_220000;66000_/LConn1 -- _CN_127261542_220000_CN_219005247_220000/LConn1 -- _CN_127261542_220000_CN_192655498_220000/LConn1
  _CN_127261542_220000_CN_127255915_220000/RConn2 -- T_127261542_220000;66000_/LConn2 -- _CN_127261542_220000_CN_219005247_220000/LConn2 -- _CN_127261542_220000_CN_192655498_220000/LConn2
  _CN_127261542_220000_CN_127255915_220000/RConn3 -- T_127261542_220000;66000_/LConn3 -- _CN_127261542_220000_CN_219005247_220000/LConn3 -- _CN_127261542_220000_CN_192655498_220000/LConn3 -- bus112/LConn1
  _CN_127261542_220000_CN_219005247_220000/RConn1 -- T_219005247_220000_/LConn1 -- _CN_219005247_220000_CN_95838096_220000/RConn1 -- _CN_219005247_220000_CN_192655498_220000/LConn1
  _CN_127261542_220000_CN_219005247_220000/RConn2 -- T_219005247_220000_/LConn2 -- _CN_219005247_220000_CN_95838096_220000/RConn2 -- _CN_219005247_220000_CN_192655498_220000/LConn2
  _CN_127261542_220000_CN_219005247_220000/RConn3 -- T_219005247_220000_/LConn3 -- _CN_219005247_220000_CN_95838096_220000/RConn3 -- bus113/LConn1 -- _CN_219005247_220000_CN_192655498_220000/LConn3
  _CN_127261542_220000_CN_192655498_220000/RConn1 -- G_192655498_/RConn1 -- _CN_219005247_220000_CN_192655498_220000/RConn1
  _CN_127261542_220000_CN_192655498_220000/RConn2 -- G_192655498_/RConn2 -- _CN_219005247_220000_CN_192655498_220000/RConn2
  _CN_127261542_220000_CN_192655498_220000/RConn3 -- G_192655498_/RConn3 -- _CN_219005247_220000_CN_192655498_220000/RConn3 -- bus114/LConn1
  _CN_131239138_220000_CN_131247022_220000/LConn1 -- T_131239138_220000_/LConn1 -- _CN_131239138_220000_CN_131236227_220000/RConn1 -- _CN_131239138_220000_CN_130782509_220000/LConn1
  _CN_131239138_220000_CN_131247022_220000/LConn2 -- T_131239138_220000_/LConn2 -- _CN_131239138_220000_CN_131236227_220000/RConn2 -- _CN_131239138_220000_CN_130782509_220000/LConn2
  _CN_131239138_220000_CN_131247022_220000/LConn3 -- T_131239138_220000_/LConn3 -- _CN_131239138_220000_CN_131236227_220000/RConn3 -- _CN_131239138_220000_CN_130782509_220000/LConn3 -- bus115/LConn1
  _CN_131239138_220000_CN_131247022_220000/RConn1 -- T_131247022_220000_/LConn1 -- _CN_131247019_220000_CN_131247022_220000/LConn1 -- _CN_131247022_220000_CN_95929780_220000/LConn1 -- _CN_219005249_220000_CN_131247022_220000/LConn1
  _CN_131239138_220000_CN_131247022_220000/RConn2 -- T_131247022_220000_/LConn2 -- _CN_131247019_220000_CN_131247022_220000/LConn2 -- _CN_131247022_220000_CN_95929780_220000/LConn2 -- _CN_219005249_220000_CN_131247022_220000/LConn2
  _CN_131239138_220000_CN_131247022_220000/RConn3 -- T_131247022_220000_/LConn3 -- _CN_131247019_220000_CN_131247022_220000/LConn3 -- _CN_131247022_220000_CN_95929780_220000/LConn3 -- bus116/LConn1 -- _CN_219005249_220000_CN_131247022_220000/LConn3
  T_130782509_220000_/LConn1 -- _CN_131239138_220000_CN_130782509_220000/RConn1
  T_130782509_220000_/LConn2 -- _CN_131239138_220000_CN_130782509_220000/RConn2
  _CN_131239138_220000_CN_130782509_220000/RConn3 -- T_130782509_220000_/LConn3 -- bus117/LConn1
  T_99772131_220000;66000_/LConn1 -- _CN_99772131_220000_CN_99788079_220000/LConn1
  T_99772131_220000;66000_/LConn2 -- _CN_99772131_220000_CN_99788079_220000/LConn2
  _CN_99772131_220000_CN_99788079_220000/LConn3 -- T_99772131_220000;66000_/LConn3 -- bus118/LConn1
  _CN_99772131_220000_CN_99788079_220000/RConn1 -- T_99788079_220000_/LConn1 -- _CN_99788079_220000_CN_213203948_220000/RConn1
  _CN_99772131_220000_CN_99788079_220000/RConn2 -- T_99788079_220000_/LConn2 -- _CN_99788079_220000_CN_213203948_220000/RConn2
  _CN_99772131_220000_CN_99788079_220000/RConn3 -- T_99788079_220000_/LConn3 -- _CN_99788079_220000_CN_213203948_220000/RConn3 -- bus119/LConn1
  T_119584035_220000;66000_/LConn1 -- _CN_119584035_220000_CN_118301256_220000/RConn1
  T_119584035_220000;66000_/LConn2 -- _CN_119584035_220000_CN_118301256_220000/RConn2
  _CN_119584035_220000_CN_118301256_220000/RConn3 -- T_119584035_220000;66000_/LConn3 -- bus120/LConn1
  G_28830169_محطة_كهرباء_شمال_القاهرة/RConn1 -- _CN_128205604_220000_CN_28830169_220000/RConn1
  G_28830169_محطة_كهرباء_شمال_القاهرة/RConn2 -- _CN_128205604_220000_CN_28830169_220000/RConn2
  _CN_128205604_220000_CN_28830169_220000/RConn3 -- G_28830169_محطة_كهرباء_شمال_القاهرة/RConn3 -- bus121/LConn1
  _CN_117393191_220000_CN_426347972_220000/LConn1 -- T_117393191_500000;220000;132000_/RConn1 -- _CN_117393191_220000_CN_93583051_220000/RConn1
  _CN_117393191_220000_CN_426347972_220000/LConn2 -- T_117393191_500000;220000;132000_/RConn2 -- _CN_117393191_220000_CN_93583051_220000/RConn2
  _CN_117393191_220000_CN_426347972_220000/LConn3 -- T_117393191_500000;220000;132000_/RConn3 -- _CN_117393191_220000_CN_93583051_220000/RConn3 -- bus122/LConn1
  _CN_117393191_220000_CN_426347972_220000/RConn1 -- T_426347972__/LConn1 -- _CN_117381489_220000_CN_426347972_220000/RConn1
  _CN_117393191_220000_CN_426347972_220000/RConn2 -- T_426347972__/LConn2 -- _CN_117381489_220000_CN_426347972_220000/RConn2
  _CN_117393191_220000_CN_426347972_220000/RConn3 -- T_426347972__/LConn3 -- _CN_117381489_220000_CN_426347972_220000/RConn3 -- bus123/LConn1
  T_219005249_220000_/LConn1 -- _CN_219005249_220000_CN_131247022_220000/RConn1
  T_219005249_220000_/LConn2 -- _CN_219005249_220000_CN_131247022_220000/RConn2
  _CN_219005249_220000_CN_131247022_220000/RConn3 -- T_219005249_220000_/LConn3 -- bus124/LConn1
  T_127398225_220000;66000_/LConn1 -- _CN_219032903_220000_CN_127398225_220000/RConn1
  T_127398225_220000;66000_/LConn2 -- _CN_219032903_220000_CN_127398225_220000/RConn2
  _CN_219032903_220000_CN_127398225_220000/RConn3 -- T_127398225_220000;66000_/LConn3 -- bus125/LConn1
  _CN_123466581_220000_CN_105569177_220000/RConn1 -- G_105569177_Abu_Sultan/RConn1 -- _CN_105694639_220000_CN_105569177_220000/RConn1 -- _CN_90608610_220000_CN_105569177_220000/RConn1
  _CN_123466581_220000_CN_105569177_220000/RConn2 -- G_105569177_Abu_Sultan/RConn2 -- _CN_105694639_220000_CN_105569177_220000/RConn2 -- _CN_90608610_220000_CN_105569177_220000/RConn2
  _CN_123466581_220000_CN_105569177_220000/RConn3 -- G_105569177_Abu_Sultan/RConn3 -- _CN_105694639_220000_CN_105569177_220000/RConn3 -- _CN_90608610_220000_CN_105569177_220000/RConn3 -- bus126/LConn1
  _CN_426156915_220000_CN_118301256_220000/RConn1 -- T_426156915__/LConn1 -- _CN_426156915_220000_CN_219716698_220000/LConn1
  _CN_426156915_220000_CN_118301256_220000/RConn2 -- T_426156915__/LConn2 -- _CN_426156915_220000_CN_219716698_220000/LConn2
  _CN_426156915_220000_CN_118301256_220000/RConn3 -- T_426156915__/LConn3 -- _CN_426156915_220000_CN_219716698_220000/LConn3 -- bus127/LConn1
  T_219716698_220000_/LConn1 -- _CN_426156915_220000_CN_219716698_220000/RConn1
  T_219716698_220000_/LConn2 -- _CN_426156915_220000_CN_219716698_220000/RConn2
  _CN_426156915_220000_CN_219716698_220000/RConn3 -- T_219716698_220000_/LConn3 -- bus128/LConn1
  G_214806696_Port_Said/RConn1 -- _CN_93650324_220000_CN_214806696_220000/RConn1
  G_214806696_Port_Said/RConn2 -- _CN_93650324_220000_CN_214806696_220000/RConn2
  _CN_93650324_220000_CN_214806696_220000/RConn3 -- G_214806696_Port_Said/RConn3 -- bus129/LConn1
  T_131247019_220000_/LConn1 -- _CN_131247019_220000_CN_131247022_220000/RConn1
  T_131247019_220000_/LConn2 -- _CN_131247019_220000_CN_131247022_220000/RConn2
  _CN_131247019_220000_CN_131247022_220000/RConn3 -- T_131247019_220000_/LConn3 -- bus130/LConn1
  G_95929780_/RConn1 -- _CN_131247022_220000_CN_95929780_220000/RConn1
  G_95929780_/RConn2 -- _CN_131247022_220000_CN_95929780_220000/RConn2
  _CN_131247022_220000_CN_95929780_220000/RConn3 -- G_95929780_/RConn3 -- bus131/LConn1
  T_131247024_220000_/LConn1 -- _CN_131247024_220000_CN_131247008_220000/LConn1
  T_131247024_220000_/LConn2 -- _CN_131247024_220000_CN_131247008_220000/LConn2
  _CN_131247024_220000_CN_131247008_220000/LConn3 -- T_131247024_220000_/LConn3 -- bus132/LConn1
  G_131247008_/RConn1 -- _CN_131247024_220000_CN_131247008_220000/RConn1
  G_131247008_/RConn2 -- _CN_131247024_220000_CN_131247008_220000/RConn2
  _CN_131247024_220000_CN_131247008_220000/RConn3 -- G_131247008_/RConn3 -- bus133/LConn1
  _CN_90608610_500000_CN_210209256_500000/LConn1 -- T_90608610_220000_/LConn1 -- _CN_90608610_500000_CN_103010149_500000/LConn1
  _CN_90608610_500000_CN_210209256_500000/LConn2 -- T_90608610_220000_/LConn2 -- _CN_90608610_500000_CN_103010149_500000/LConn2
  _CN_90608610_500000_CN_210209256_500000/LConn3 -- T_90608610_220000_/LConn3 -- _CN_90608610_500000_CN_103010149_500000/LConn3 -- bus134/LConn1
  _CN_90608610_500000_CN_210209256_500000/RConn1 -- T_210209256_500000_/LConn1 -- _CN_210209256_500000_CN_97721460_500000/LConn1
  _CN_90608610_500000_CN_210209256_500000/RConn2 -- T_210209256_500000_/LConn2 -- _CN_210209256_500000_CN_97721460_500000/LConn2
  _CN_90608610_500000_CN_210209256_500000/RConn3 -- T_210209256_500000_/LConn3 -- _CN_210209256_500000_CN_97721460_500000/LConn3 -- bus135/LConn1
  _CN_90608610_500000_CN_103010149_500000/RConn1 -- T_103010149_500000_/LConn1 -- _CN_103010149_500000_CN_427608566_500000/LConn1 -- _CN_128205604_500000_CN_103010149_500000/LConn1
  _CN_90608610_500000_CN_103010149_500000/RConn2 -- T_103010149_500000_/LConn2 -- _CN_103010149_500000_CN_427608566_500000/LConn2 -- _CN_128205604_500000_CN_103010149_500000/LConn2
  _CN_90608610_500000_CN_103010149_500000/RConn3 -- T_103010149_500000_/LConn3 -- _CN_103010149_500000_CN_427608566_500000/LConn3 -- bus136/LConn1 -- _CN_128205604_500000_CN_103010149_500000/LConn3
  _CN_218893323_500000_CN_128205604_500000/LConn1 -- T_218893323_500000;220000_Cairo_West_Substation/LConn1 -- _CN_218893323_500000_CN_218972673_500000/LConn1
  _CN_218893323_500000_CN_128205604_500000/LConn2 -- T_218893323_500000;220000_Cairo_West_Substation/LConn2 -- _CN_218893323_500000_CN_218972673_500000/LConn2
  _CN_218893323_500000_CN_128205604_500000/LConn3 -- T_218893323_500000;220000_Cairo_West_Substation/LConn3 -- _CN_218893323_500000_CN_218972673_500000/LConn3 -- bus137/LConn1
  _CN_218893323_500000_CN_128205604_500000/RConn1 -- T_128205604_500000_/LConn1 -- _CN_128205604_500000_CN_103010149_500000/RConn1
  _CN_218893323_500000_CN_128205604_500000/RConn2 -- T_128205604_500000_/LConn2 -- _CN_128205604_500000_CN_103010149_500000/RConn2
  _CN_218893323_500000_CN_128205604_500000/RConn3 -- T_128205604_500000_/LConn3 -- _CN_128205604_500000_CN_103010149_500000/RConn3 -- bus138/LConn1
  G_218972673_/RConn1 -- _CN_218893323_500000_CN_218972673_500000/RConn1
  G_218972673_/RConn2 -- _CN_218893323_500000_CN_218972673_500000/RConn2
  _CN_218893323_500000_CN_218972673_500000/RConn3 -- G_218972673_/RConn3 -- bus139/LConn1
  _CN_103010149_500000_CN_427608566_500000/RConn1 -- T_427608566__/LConn1 -- _CN_118310545_500000_CN_427608566_500000/LConn1
  _CN_103010149_500000_CN_427608566_500000/RConn2 -- T_427608566__/LConn2 -- _CN_118310545_500000_CN_427608566_500000/LConn2
  _CN_103010149_500000_CN_427608566_500000/RConn3 -- T_427608566__/LConn3 -- _CN_118310545_500000_CN_427608566_500000/LConn3 -- bus140/LConn1
  T_426998278__/LConn1 -- _CN_426998278_500000_CN_115491527_500000/LConn1
  T_426998278__/LConn2 -- _CN_426998278_500000_CN_115491527_500000/LConn2
  _CN_426998278_500000_CN_115491527_500000/LConn3 -- T_426998278__/LConn3 -- bus141/LConn1
  _CN_426998278_500000_CN_115491527_500000/RConn1 -- T_115491527_500000;220000;132000_/LConn1 -- _CN_117393191_500000_CN_115491527_500000/LConn1
  _CN_426998278_500000_CN_115491527_500000/RConn2 -- T_115491527_500000;220000;132000_/LConn2 -- _CN_117393191_500000_CN_115491527_500000/LConn2
  _CN_426998278_500000_CN_115491527_500000/RConn3 -- T_115491527_500000;220000;132000_/LConn3 -- _CN_117393191_500000_CN_115491527_500000/LConn3 -- bus142/LConn1
  T_117393191_500000;220000;132000_/LConn1 -- _CN_117393191_500000_CN_115491527_500000/RConn1
  T_117393191_500000;220000;132000_/LConn2 -- _CN_117393191_500000_CN_115491527_500000/RConn2
  _CN_117393191_500000_CN_115491527_500000/RConn3 -- T_117393191_500000;220000;132000_/LConn3 -- bus143/LConn1
  _CN_210209256_500000_CN_97721460_500000/RConn1 -- T_97721460_220000_/LConn1 -- _CN_97721460_500000_CN_120204568_500000/LConn1
  _CN_210209256_500000_CN_97721460_500000/RConn2 -- T_97721460_220000_/LConn2 -- _CN_97721460_500000_CN_120204568_500000/LConn2
  _CN_210209256_500000_CN_97721460_500000/RConn3 -- T_97721460_220000_/LConn3 -- _CN_97721460_500000_CN_120204568_500000/LConn3 -- bus144/LConn1
  T_218972674__/LConn1 -- _CN_218972674_500000_CN_131236227_220000/RConn1
  T_218972674__/LConn2 -- _CN_218972674_500000_CN_131236227_220000/RConn2
  _CN_218972674_500000_CN_131236227_220000/RConn3 -- T_218972674__/LConn3 -- bus145/LConn1
  _CN_118310545_500000_CN_118301256_220000/RConn1 -- T_118310545_500000;220000_/LConn1 -- _CN_118310545_500000_CN_427608566_500000/RConn1
  _CN_118310545_500000_CN_118301256_220000/RConn2 -- T_118310545_500000;220000_/LConn2 -- _CN_118310545_500000_CN_427608566_500000/RConn2
  _CN_118310545_500000_CN_118301256_220000/RConn3 -- T_118310545_500000;220000_/LConn3 -- _CN_118310545_500000_CN_427608566_500000/RConn3 -- bus146/LConn1
  T_120204568__/LConn1 -- _CN_97721460_500000_CN_120204568_500000/RConn1
  T_120204568__/LConn2 -- _CN_97721460_500000_CN_120204568_500000/RConn2
  _CN_97721460_500000_CN_120204568_500000/RConn3 -- T_120204568__/LConn3 -- bus147/LConn1
  T_426825819__/RConn1 -- L_426825819/LConn1
  T_426825819__/RConn2 -- L_426825819/LConn2
  L_426825819/LConn3 -- T_426825819__/RConn3 -- bus148/LConn1
  T_102788377_132000;66000_/RConn1 -- L_102788377/LConn1
  T_102788377_132000;66000_/RConn2 -- L_102788377/LConn2
  L_102788377/LConn3 -- T_102788377_132000;66000_/RConn3 -- bus149/LConn1
  T_112984533_132000_/RConn1 -- L_112984533/LConn1
  T_112984533_132000_/RConn2 -- L_112984533/LConn2
  L_112984533/LConn3 -- T_112984533_132000_/RConn3 -- bus150/LConn1
  T_113004375_132000_/RConn1 -- L_113004375/LConn1
  T_113004375_132000_/RConn2 -- L_113004375/LConn2
  L_113004375/LConn3 -- T_113004375_132000_/RConn3 -- bus151/LConn1
  T_219583075_132000_/RConn1 -- L_219583075/LConn1
  T_219583075_132000_/RConn2 -- L_219583075/LConn2
  L_219583075/LConn3 -- T_219583075_132000_/RConn3 -- bus152/LConn1
  T_263541774__/RConn1 -- L_263541774/LConn1
  T_263541774__/RConn2 -- L_263541774/LConn2
  L_263541774/LConn3 -- T_263541774__/RConn3 -- bus153/LConn1
  T_263541777__/RConn1 -- L_263541777/LConn1
  T_263541777__/RConn2 -- L_263541777/LConn2
  L_263541777/LConn3 -- T_263541777__/RConn3 -- bus154/LConn1
  T_117328910__/RConn1 -- L_117328910/LConn1
  T_117328910__/RConn2 -- L_117328910/LConn2
  L_117328910/LConn3 -- T_117328910__/RConn3 -- bus155/LConn1
  T_213203947_132000;66000_/RConn1 -- L_213203947/LConn1
  T_213203947_132000;66000_/RConn2 -- L_213203947/LConn2
  L_213203947/LConn3 -- T_213203947_132000;66000_/RConn3 -- bus156/LConn1
  T_130440397_132000_/RConn1 -- L_130440397/LConn1
  T_130440397_132000_/RConn2 -- L_130440397/LConn2
  L_130440397/LConn3 -- T_130440397_132000_/RConn3 -- bus157/LConn1
  T_130440404_132000_/RConn1 -- L_130440404/LConn1
  T_130440404_132000_/RConn2 -- L_130440404/LConn2
  L_130440404/LConn3 -- T_130440404_132000_/RConn3 -- bus158/LConn1
  T_230637780_132000_/RConn1 -- L_230637780/LConn1
  T_230637780_132000_/RConn2 -- L_230637780/LConn2
  L_230637780/LConn3 -- T_230637780_132000_/RConn3 -- bus159/LConn1
  T_116612828_220000_/RConn1 -- L_116612828/LConn1
  T_116612828_220000_/RConn2 -- L_116612828/LConn2
  L_116612828/LConn3 -- T_116612828_220000_/RConn3 -- bus160/LConn1
  T_130435119_220000;66000_/RConn1 -- L_130435119/LConn1
  T_130435119_220000;66000_/RConn2 -- L_130435119/LConn2
  L_130435119/LConn3 -- T_130435119_220000;66000_/RConn3 -- bus161/LConn1
  T_263290997_220000;66000_/RConn1 -- L_263290997/LConn1
  T_263290997_220000;66000_/RConn2 -- L_263290997/LConn2
  L_263290997/LConn3 -- T_263290997_220000;66000_/RConn3 -- bus162/LConn1
  T_128182735_220000_/RConn1 -- L_128182735/LConn1
  T_128182735_220000_/RConn2 -- L_128182735/LConn2
  L_128182735/LConn3 -- T_128182735_220000_/RConn3 -- bus163/LConn1
  T_98390022_220000;66000_/RConn1 -- L_98390022/LConn1
  T_98390022_220000;66000_/RConn2 -- L_98390022/LConn2
  L_98390022/LConn3 -- T_98390022_220000;66000_/RConn3 -- bus164/LConn1
  T_93650324_220000_/RConn1 -- L_93650324/LConn1
  T_93650324_220000_/RConn2 -- L_93650324/LConn2
  L_93650324/LConn3 -- T_93650324_220000_/RConn3 -- bus165/LConn1
  T_128123911_220000_/RConn1 -- L_128123911/LConn1
  T_128123911_220000_/RConn2 -- L_128123911/LConn2
  L_128123911/LConn3 -- T_128123911_220000_/RConn3 -- bus166/LConn1
  T_127255915_220000;66000_/RConn1 -- L_127255915/LConn1
  T_127255915_220000;66000_/RConn2 -- L_127255915/LConn2
  L_127255915/LConn3 -- T_127255915_220000;66000_/RConn3 -- bus167/LConn1
  T_103998472_220000_/RConn1 -- L_103998472/LConn1
  T_103998472_220000_/RConn2 -- L_103998472/LConn2
  L_103998472/LConn3 -- T_103998472_220000_/RConn3 -- bus168/LConn1
  T_126503845_220000;132000_/RConn1 -- L_126503845/LConn1
  T_126503845_220000;132000_/RConn2 -- L_126503845/LConn2
  L_126503845/LConn3 -- T_126503845_220000;132000_/RConn3 -- bus169/LConn1
  T_213211662_220000_/RConn1 -- L_213211662/LConn1
  T_213211662_220000_/RConn2 -- L_213211662/LConn2
  L_213211662/LConn3 -- T_213211662_220000_/RConn3 -- bus170/LConn1
  T_130229777_220000;66000_/RConn1 -- L_130229777/LConn1
  T_130229777_220000;66000_/RConn2 -- L_130229777/LConn2
  L_130229777/LConn3 -- T_130229777_220000;66000_/RConn3 -- bus171/LConn1
  T_216227836_220000_/RConn1 -- L_216227836/LConn1
  T_216227836_220000_/RConn2 -- L_216227836/LConn2
  L_216227836/LConn3 -- T_216227836_220000_/RConn3 -- bus172/LConn1
  T_97702932_220000_/RConn1 -- L_97702932/LConn1
  T_97702932_220000_/RConn2 -- L_97702932/LConn2
  L_97702932/LConn3 -- T_97702932_220000_/RConn3 -- bus173/LConn1
  T_219687981_220000_/RConn1 -- L_219687981/LConn1
  T_219687981_220000_/RConn2 -- L_219687981/LConn2
  L_219687981/LConn3 -- T_219687981_220000_/RConn3 -- bus174/LConn1
  T_130572646_220000_/RConn1 -- L_130572646/LConn1
  T_130572646_220000_/RConn2 -- L_130572646/LConn2
  L_130572646/LConn3 -- T_130572646_220000_/RConn3 -- bus175/LConn1
  T_214809518_220000_/RConn1 -- L_214809518/LConn1
  T_214809518_220000_/RConn2 -- L_214809518/LConn2
  L_214809518/LConn3 -- T_214809518_220000_/RConn3 -- bus176/LConn1
  T_216093003_220000_/RConn1 -- L_216093003/LConn1
  T_216093003_220000_/RConn2 -- L_216093003/LConn2
  L_216093003/LConn3 -- T_216093003_220000_/RConn3 -- bus177/LConn1
  T_276511906_220000;66000_/RConn1 -- L_276511906/LConn1
  T_276511906_220000;66000_/RConn2 -- L_276511906/LConn2
  L_276511906/LConn3 -- T_276511906_220000;66000_/RConn3 -- bus178/LConn1
  T_216214039_220000_/RConn1 -- L_216214039/LConn1
  T_216214039_220000_/RConn2 -- L_216214039/LConn2
  L_216214039/LConn3 -- T_216214039_220000_/RConn3 -- bus179/LConn1
  T_343022340_220000_/RConn1 -- L_343022340/LConn1
  T_343022340_220000_/RConn2 -- L_343022340/LConn2
  L_343022340/LConn3 -- T_343022340_220000_/RConn3 -- bus180/LConn1
  T_219020313_220000_/RConn1 -- L_219020313/LConn1
  T_219020313_220000_/RConn2 -- L_219020313/LConn2
  L_219020313/LConn3 -- T_219020313_220000_/RConn3 -- bus181/LConn1
  T_219032903_220000_/RConn1 -- L_219032903/LConn1
  T_219032903_220000_/RConn2 -- L_219032903/LConn2
  L_219032903/LConn3 -- T_219032903_220000_/RConn3 -- bus182/LConn1
  T_119907869_220000_/RConn1 -- L_119907869/LConn1
  T_119907869_220000_/RConn2 -- L_119907869/LConn2
  L_119907869/LConn3 -- T_119907869_220000_/RConn3 -- bus183/LConn1
  T_427608567__/RConn1 -- L_427608567/LConn1
  T_427608567__/RConn2 -- L_427608567/LConn2
  L_427608567/LConn3 -- T_427608567__/RConn3 -- bus184/LConn1
  T_119907603_220000_/RConn1 -- L_119907603/LConn1
  T_119907603_220000_/RConn2 -- L_119907603/LConn2
  L_119907603/LConn3 -- T_119907603_220000_/RConn3 -- bus185/LConn1
  T_92878367_220000_/RConn1 -- L_92878367/LConn1
  T_92878367_220000_/RConn2 -- L_92878367/LConn2
  L_92878367/LConn3 -- T_92878367_220000_/RConn3 -- bus186/LConn1
  T_105191630_220000;66000_/RConn1 -- L_105191630/LConn1
  T_105191630_220000;66000_/RConn2 -- L_105191630/LConn2
  L_105191630/LConn3 -- T_105191630_220000;66000_/RConn3 -- bus187/LConn1
  T_119909663_220000_/RConn1 -- L_119909663/LConn1
  T_119909663_220000_/RConn2 -- L_119909663/LConn2
  L_119909663/LConn3 -- T_119909663_220000_/RConn3 -- bus188/LConn1
  T_98663458_220000;66000_/RConn1 -- L_98663458/LConn1
  T_98663458_220000;66000_/RConn2 -- L_98663458/LConn2
  L_98663458/LConn3 -- T_98663458_220000;66000_/RConn3 -- bus189/LConn1
  T_98663507_220000;66000_/RConn1 -- L_98663507/LConn1
  T_98663507_220000;66000_/RConn2 -- L_98663507/LConn2
  L_98663507/LConn3 -- T_98663507_220000;66000_/RConn3 -- bus190/LConn1
  T_128125479_220000_/RConn1 -- L_128125479/LConn1
  T_128125479_220000_/RConn2 -- L_128125479/LConn2
  L_128125479/LConn3 -- T_128125479_220000_/RConn3 -- bus191/LConn1
  T_128129616_220000_/RConn1 -- L_128129616/LConn1
  T_128129616_220000_/RConn2 -- L_128129616/LConn2
  L_128129616/LConn3 -- T_128129616_220000_/RConn3 -- bus192/LConn1
  T_219583071_220000;66000_/RConn1 -- L_219583071/LConn1
  T_219583071_220000;66000_/RConn2 -- L_219583071/LConn2
  L_219583071/LConn3 -- T_219583071_220000;66000_/RConn3 -- bus193/LConn1
  T_219295621_220000_/RConn1 -- L_219295621/LConn1
  T_219295621_220000_/RConn2 -- L_219295621/LConn2
  L_219295621/LConn3 -- T_219295621_220000_/RConn3 -- bus194/LConn1
  T_426596409_220000_/RConn1 -- L_426596409/LConn1
  T_426596409_220000_/RConn2 -- L_426596409/LConn2
  L_426596409/LConn3 -- T_426596409_220000_/RConn3 -- bus195/LConn1
  T_117342821_220000_/RConn1 -- L_117342821/LConn1
  T_117342821_220000_/RConn2 -- L_117342821/LConn2
  L_117342821/LConn3 -- T_117342821_220000_/RConn3 -- bus196/LConn1
  T_426825830_220000_/RConn1 -- L_426825830/LConn1
  T_426825830_220000_/RConn2 -- L_426825830/LConn2
  L_426825830/LConn3 -- T_426825830_220000_/RConn3 -- bus197/LConn1
  T_120521277__/RConn1 -- L_120521277/LConn1
  T_120521277__/RConn2 -- L_120521277/LConn2
  L_120521277/LConn3 -- T_120521277__/RConn3 -- bus198/LConn1
  T_120516781__/RConn1 -- L_120516781/LConn1
  T_120516781__/RConn2 -- L_120516781/LConn2
  L_120516781/LConn3 -- T_120516781__/RConn3 -- bus199/LConn1
  T_123223445_220000;66000_/RConn1 -- L_123223445/LConn1
  T_123223445_220000;66000_/RConn2 -- L_123223445/LConn2
  L_123223445/LConn3 -- T_123223445_220000;66000_/RConn3 -- bus200/LConn1
  T_122132699_220000;66000_/RConn1 -- L_122132699/LConn1
  T_122132699_220000;66000_/RConn2 -- L_122132699/LConn2
  L_122132699/LConn3 -- T_122132699_220000;66000_/RConn3 -- bus201/LConn1
  T_117528642_220000;66000_/RConn1 -- L_117528642/LConn1
  T_117528642_220000;66000_/RConn2 -- L_117528642/LConn2
  L_117528642/LConn3 -- T_117528642_220000;66000_/RConn3 -- bus202/LConn1
  T_218898508_220000;66000_/RConn1 -- L_218898508/LConn1
  T_218898508_220000;66000_/RConn2 -- L_218898508/LConn2
  L_218898508/LConn3 -- T_218898508_220000;66000_/RConn3 -- bus203/LConn1
  T_126280786_220000;66000_/RConn1 -- L_126280786/LConn1
  T_126280786_220000;66000_/RConn2 -- L_126280786/LConn2
  L_126280786/LConn3 -- T_126280786_220000;66000_/RConn3 -- bus204/LConn1
  T_265751903__/RConn1 -- L_265751903/LConn1
  T_265751903__/RConn2 -- L_265751903/LConn2
  L_265751903/LConn3 -- T_265751903__/RConn3 -- bus205/LConn1
  T_126200917_220000_/RConn1 -- L_126200917/LConn1
  T_126200917_220000_/RConn2 -- L_126200917/LConn2
  L_126200917/LConn3 -- T_126200917_220000_/RConn3 -- bus206/LConn1
  T_117671808_220000_/RConn1 -- L_117671808/LConn1
  T_117671808_220000_/RConn2 -- L_117671808/LConn2
  L_117671808/LConn3 -- T_117671808_220000_/RConn3 -- bus207/LConn1
  T_218975834_220000_/RConn1 -- L_218975834/LConn1
  T_218975834_220000_/RConn2 -- L_218975834/LConn2
  L_218975834/LConn3 -- T_218975834_220000_/RConn3 -- bus208/LConn1
  T_218976990_220000_/RConn1 -- L_218976990/LConn1
  T_218976990_220000_/RConn2 -- L_218976990/LConn2
  L_218976990/LConn3 -- T_218976990_220000_/RConn3 -- bus209/LConn1
  T_216224349__Zafarana_7/RConn1 -- L_216224349/LConn1
  T_216224349__Zafarana_7/RConn2 -- L_216224349/LConn2
  L_216224349/LConn3 -- T_216224349__Zafarana_7/RConn3 -- bus210/LConn1
  T_130572645__Zafarana_7/RConn1 -- L_130572645/LConn1
  T_130572645__Zafarana_7/RConn2 -- L_130572645/LConn2
  L_130572645/LConn3 -- T_130572645__Zafarana_7/RConn3 -- bus211/LConn1
  T_427596550__El_Zayt_wind_farm/RConn1 -- L_427596550/LConn1
  T_427596550__El_Zayt_wind_farm/RConn2 -- L_427596550/LConn2
  L_427596550/LConn3 -- T_427596550__El_Zayt_wind_farm/RConn3 -- bus212/LConn1
  T_103015033_220000;66000_/RConn1 -- L_103015033/LConn1
  T_103015033_220000;66000_/RConn2 -- L_103015033/LConn2
  L_103015033/LConn3 -- T_103015033_220000;66000_/RConn3 -- bus213/LConn1
  T_117381489_220000;66000_/RConn1 -- L_117381489/LConn1
  T_117381489_220000;66000_/RConn2 -- L_117381489/LConn2
  L_117381489/LConn3 -- T_117381489_220000;66000_/RConn3 -- bus214/LConn1
  T_97721447_220000;66000_/RConn1 -- L_97721447/LConn1
  T_97721447_220000;66000_/RConn2 -- L_97721447/LConn2
  L_97721447/LConn3 -- T_97721447_220000;66000_/RConn3 -- bus215/LConn1
  T_176719989_220000;66000_/RConn1 -- L_176719989/LConn1
  T_176719989_220000;66000_/RConn2 -- L_176719989/LConn2
  L_176719989/LConn3 -- T_176719989_220000;66000_/RConn3 -- bus216/LConn1
  T_93714538_220000_/RConn1 -- L_93714538/LConn1
  T_93714538_220000_/RConn2 -- L_93714538/LConn2
  L_93714538/LConn3 -- T_93714538_220000_/RConn3 -- bus217/LConn1
  T_105694639_220000_/RConn1 -- L_105694639/LConn1
  T_105694639_220000_/RConn2 -- L_105694639/LConn2
  L_105694639/LConn3 -- T_105694639_220000_/RConn3 -- bus218/LConn1
  T_123466581_220000;66000_/RConn1 -- L_123466581/LConn1
  T_123466581_220000;66000_/RConn2 -- L_123466581/LConn2
  L_123466581/LConn3 -- T_123466581_220000;66000_/RConn3 -- bus219/LConn1
  T_127243911_220000;66000_/RConn1 -- L_127243911/LConn1
  T_127243911_220000;66000_/RConn2 -- L_127243911/LConn2
  L_127243911/LConn3 -- T_127243911_220000;66000_/RConn3 -- bus220/LConn1
  T_97852047_220000_/RConn1 -- L_97852047/LConn1
  T_97852047_220000_/RConn2 -- L_97852047/LConn2
  L_97852047/LConn3 -- T_97852047_220000_/RConn3 -- bus221/LConn1
  T_118345956_220000_/RConn1 -- L_118345956/LConn1
  T_118345956_220000_/RConn2 -- L_118345956/LConn2
  L_118345956/LConn3 -- T_118345956_220000_/RConn3 -- bus222/LConn1
  T_419686238__/RConn1 -- L_419686238/LConn1
  T_419686238__/RConn2 -- L_419686238/LConn2
  L_419686238/LConn3 -- T_419686238__/RConn3 -- bus223/LConn1
  T_102988954_220000_/RConn1 -- L_102988954/LConn1
  T_102988954_220000_/RConn2 -- L_102988954/LConn2
  L_102988954/LConn3 -- T_102988954_220000_/RConn3 -- bus224/LConn1
  T_102988963_220000_/RConn1 -- L_102988963/LConn1
  T_102988963_220000_/RConn2 -- L_102988963/LConn2
  L_102988963/LConn3 -- T_102988963_220000_/RConn3 -- bus225/LConn1
  T_122238112_220000;66000_/RConn1 -- L_122238112/LConn1
  T_122238112_220000;66000_/RConn2 -- L_122238112/LConn2
  L_122238112/LConn3 -- T_122238112_220000;66000_/RConn3 -- bus226/LConn1
  T_120516782_220000_/RConn1 -- L_120516782/LConn1
  T_120516782_220000_/RConn2 -- L_120516782/LConn2
  L_120516782/LConn3 -- T_120516782_220000_/RConn3 -- bus227/LConn1
  T_93699965_220000;66000_/RConn1 -- L_93699965/LConn1
  T_93699965_220000;66000_/RConn2 -- L_93699965/LConn2
  L_93699965/LConn3 -- T_93699965_220000;66000_/RConn3 -- bus228/LConn1
  T_426156916__/RConn1 -- L_426156916/LConn1
  T_426156916__/RConn2 -- L_426156916/LConn2
  L_426156916/LConn3 -- T_426156916__/RConn3 -- bus229/LConn1
  T_94566888_220000;66000_/RConn1 -- L_94566888/LConn1
  T_94566888_220000;66000_/RConn2 -- L_94566888/LConn2
  L_94566888/LConn3 -- T_94566888_220000;66000_/RConn3 -- bus230/LConn1
  T_218980895_220000_/RConn1 -- L_218980895/LConn1
  T_218980895_220000_/RConn2 -- L_218980895/LConn2
  L_218980895/LConn3 -- T_218980895_220000_/RConn3 -- bus231/LConn1
  T_218983235_220000_/RConn1 -- L_218983235/LConn1
  T_218983235_220000_/RConn2 -- L_218983235/LConn2
  L_218983235/LConn3 -- T_218983235_220000_/RConn3 -- bus232/LConn1
  T_263365083__/RConn1 -- L_263365083/LConn1
  T_263365083__/RConn2 -- L_263365083/LConn2
  L_263365083/LConn3 -- T_263365083__/RConn3 -- bus233/LConn1
  T_130524402_220000_/RConn1 -- L_130524402/LConn1
  T_130524402_220000_/RConn2 -- L_130524402/LConn2
  L_130524402/LConn3 -- T_130524402_220000_/RConn3 -- bus234/LConn1
  T_99494604_220000_/RConn1 -- L_99494604/LConn1
  T_99494604_220000_/RConn2 -- L_99494604/LConn2
  L_99494604/LConn3 -- T_99494604_220000_/RConn3 -- bus235/LConn1
  T_427790093__/RConn1 -- L_427790093/LConn1
  T_427790093__/RConn2 -- L_427790093/LConn2
  L_427790093/LConn3 -- T_427790093__/RConn3 -- bus236/LConn1
  T_127261542_220000;66000_/RConn1 -- L_127261542/LConn1
  T_127261542_220000;66000_/RConn2 -- L_127261542/LConn2
  L_127261542/LConn3 -- T_127261542_220000;66000_/RConn3 -- bus237/LConn1
  T_219005247_220000_/RConn1 -- L_219005247/LConn1
  T_219005247_220000_/RConn2 -- L_219005247/LConn2
  L_219005247/LConn3 -- T_219005247_220000_/RConn3 -- bus238/LConn1
  T_131239138_220000_/RConn1 -- L_131239138/LConn1
  T_131239138_220000_/RConn2 -- L_131239138/LConn2
  L_131239138/LConn3 -- T_131239138_220000_/RConn3 -- bus239/LConn1
  T_131247022_220000_/RConn1 -- L_131247022/LConn1
  T_131247022_220000_/RConn2 -- L_131247022/LConn2
  L_131247022/LConn3 -- T_131247022_220000_/RConn3 -- bus240/LConn1
  T_130782509_220000_/RConn1 -- L_130782509/LConn1
  T_130782509_220000_/RConn2 -- L_130782509/LConn2
  L_130782509/LConn3 -- T_130782509_220000_/RConn3 -- bus241/LConn1
  T_99772131_220000;66000_/RConn1 -- L_99772131/LConn1
  T_99772131_220000;66000_/RConn2 -- L_99772131/LConn2
  L_99772131/LConn3 -- T_99772131_220000;66000_/RConn3 -- bus242/LConn1
  T_99788079_220000_/RConn1 -- L_99788079/LConn1
  T_99788079_220000_/RConn2 -- L_99788079/LConn2
  L_99788079/LConn3 -- T_99788079_220000_/RConn3 -- bus243/LConn1
  T_119584035_220000;66000_/RConn1 -- L_119584035/LConn1
  T_119584035_220000;66000_/RConn2 -- L_119584035/LConn2
  L_119584035/LConn3 -- T_119584035_220000;66000_/RConn3 -- bus244/LConn1
  T_426347972__/RConn1 -- L_426347972/LConn1
  T_426347972__/RConn2 -- L_426347972/LConn2
  L_426347972/LConn3 -- T_426347972__/RConn3 -- bus245/LConn1
  T_219005249_220000_/RConn1 -- L_219005249/LConn1
  T_219005249_220000_/RConn2 -- L_219005249/LConn2
  L_219005249/LConn3 -- T_219005249_220000_/RConn3 -- bus246/LConn1
  T_127398225_220000;66000_/RConn1 -- L_127398225/LConn1
  T_127398225_220000;66000_/RConn2 -- L_127398225/LConn2
  L_127398225/LConn3 -- T_127398225_220000;66000_/RConn3 -- bus247/LConn1
  T_426156915__/RConn1 -- L_426156915/LConn1
  T_426156915__/RConn2 -- L_426156915/LConn2
  L_426156915/LConn3 -- T_426156915__/RConn3 -- bus248/LConn1
  T_219716698_220000_/RConn1 -- L_219716698/LConn1
  T_219716698_220000_/RConn2 -- L_219716698/LConn2
  L_219716698/LConn3 -- T_219716698_220000_/RConn3 -- bus249/LConn1
  T_131247019_220000_/RConn1 -- L_131247019/LConn1
  T_131247019_220000_/RConn2 -- L_131247019/LConn2
  L_131247019/LConn3 -- T_131247019_220000_/RConn3 -- bus250/LConn1
  T_131247024_220000_/RConn1 -- L_131247024/LConn1
  T_131247024_220000_/RConn2 -- L_131247024/LConn2
  L_131247024/LConn3 -- T_131247024_220000_/RConn3 -- bus251/LConn1
  T_210209256_500000_/RConn1 -- L_210209256/LConn1
  T_210209256_500000_/RConn2 -- L_210209256/LConn2
  L_210209256/LConn3 -- T_210209256_500000_/RConn3 -- bus252/LConn1
  T_218893323_500000;220000_Cairo_West_Substation/RConn1 -- L_218893323/LConn1
  T_218893323_500000;220000_Cairo_West_Substation/RConn2 -- L_218893323/LConn2
  L_218893323/LConn3 -- T_218893323_500000;220000_Cairo_West_Substation/RConn3 -- bus253/LConn1
  T_427608566__/RConn1 -- L_427608566/LConn1
  T_427608566__/RConn2 -- L_427608566/LConn2
  L_427608566/LConn3 -- T_427608566__/RConn3 -- bus254/LConn1
  T_426998278__/RConn1 -- L_426998278/LConn1
  T_426998278__/RConn2 -- L_426998278/LConn2
  L_426998278/LConn3 -- T_426998278__/RConn3 -- bus255/LConn1
  T_120204568__/RConn1 -- L_120204568/LConn1
  T_120204568__/RConn2 -- L_120204568/LConn2
  L_120204568/LConn3 -- T_120204568__/RConn3 -- bus256/LConn1
